simulink model "section4_simulation_editedbyzym"  (R2023b)
settings: Solver=FixedStepAuto  StartTime=0.0  StopTime=620  FixedStep=0.001  RelTol=1e-3
(part 1 of 2)
settings Model: PacingRate=100  Creator=DELL  LastModifiedBy=Administrator
settings SolverCC: AlgebraicLoopSolver=TrustRegion
settings OptimizationCC: EnhancedBackFolding=on  PassReuseOutputArgsThreshold=0  MaxStackSize=64  OptimizeBlockOrder=speed  DifferentSizesBufferReuse=on  OptimizationCustomize=off
settings DebuggingCC: ParameterTunabilityLossMsg=error  UnconnectedInputMsg=warning  UnconnectedOutputMsg=warning  UnconnectedLineMsg=warning  ArithmeticOperatorsInVariantConditions=warning
settings HardwareCC: ProdBitPerPointer=32  ProdBitPerSizeT=32  ProdBitPerPtrDiffT=32  ProdLargestAtomicFloat=None  ProdIntDivRoundTo=Undefined  ProdEndianess=Unspecified  ProdWordSize=32  ProdHWDeviceType=Generic->Unspecified (assume 32-bit Generic)
settings ModelReferenceCC: EnableRefExpFcnMdlSchedulingChecks=on
settings SFSimCC: MATLABDynamicMemAlloc=off  CustomCodeUndefinedFunction=UseInterfaceOnly
settings RTWCC: Toolchain=Catkin
settings CodeAppCC: ForceParamTrailComments=on  OperatorAnnotations=on
settings GRTTargetCC: TargetLangStandard=C89/C90 (ANSI)

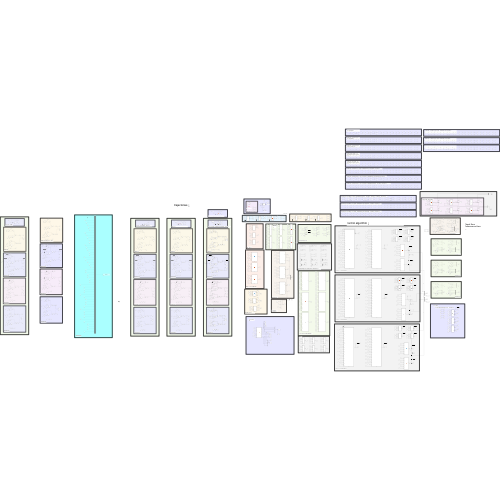
[thumbnail: Simulink's stored preview of the top-level diagram]
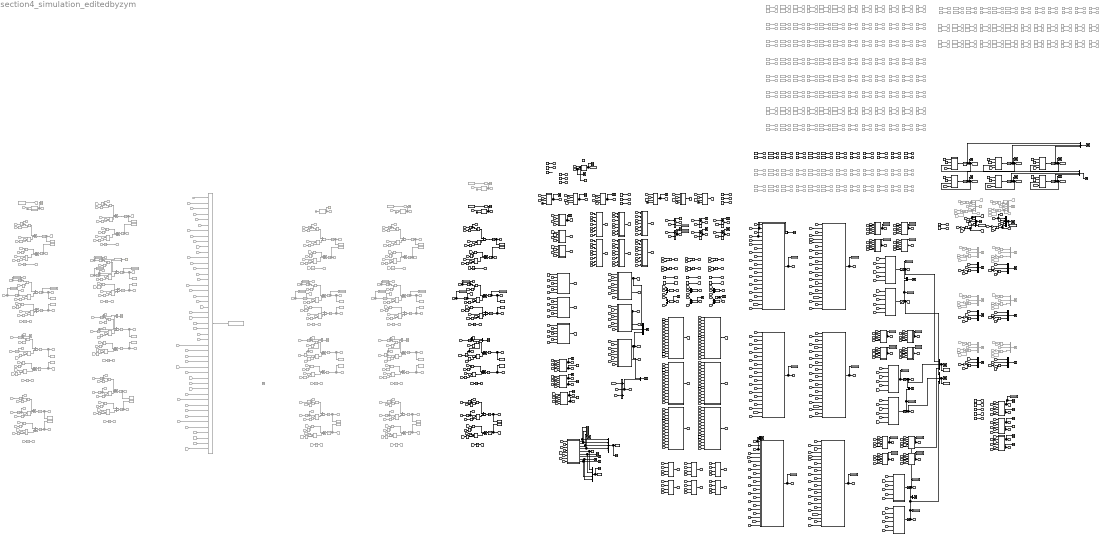
== system section4_simulation_editedbyzym ==
  note: 自适应律（6字工况）
  note: 一元二次方程中tauL和tauR的系数
  note: 控制器参数（ 固定rphi23，步长0.001,3车撞界且角度误差有稳态误差 ）
  note: dotz √
  note: 反步法新建误差delta1和delta2 √
  note: dot ei
      | √
  note: z(t)=e(t)/rou(t),并给出z(t)的上限及下限的绝对值 √
  note: 动力学模块
  note: rPHIji
  note: rdji
  note: ei 距离和角度误差√
  note: phiji,arfji（4.5）√
  note: dji（4.5）√
  note: dot,dji 三个从车的dji导数√
  note: dot,arfji,phiji √
  note: 控制器设计（1）Controller of Robot 1
  note: 预设性能对比1
  note: 预设性能对比2
  note: 预设性能对比3
  note: 预设性能对比
  note: Toworkspace
  note: 小车的转动惯量用圆柱模型来估算；J=1/2*M*L^2
  note: 我猜是队形设置，即理想间距和角度
      | 原文中（3.71）
  note: rphi23由计算得到（4.5）
  note: 为何dphi23有一个额外的修正？
  note: 编队距离和角度参数
  note: 预设性能函数
  note: 控制器设计（2） Controller of Robot 2
  note: 控制器设计（3） Controller of Robot 3
  note: leader运动学模型 原文（2.6）
  note: follower1模型
  note: follower3模型
  note: follower2模型
  note: 控制器参数（步长0.001,3车撞界且角度误差有稳态误差）
  note: follower3模型
  note: follower1模型
  note: follower2模型
  note: leader模型
  note: 6字型工况（调试）
  note: 控制器参数(固定rphi23，步长0.001,3车撞界且角度误差有稳态误差)
  note: follower3模型
  note: follower1模型
  note: follower2模型
  note: leader模型
  note: 6字工况改丝带工况t=620（从直线调试，成功运行）
  note: 控制器参数（步长0.001,直线工况收敛，lowz3p=20）
  note: 控制器参数（步长0.001,直线工况收敛，lowz3p=50）
  note: 控制器参数（步长0.001,直线工况收敛，lowz3p=50,力矩双向限幅10）
  note: 控制器参数（步长0.001,直线工况收敛，lowz3p=50,力矩双向限幅5）
  note: 控制器参数（步长0.001,直线工况收敛，lowz3p=50,力矩双向限幅2.5）
  note: 控制器参数（步长0.001,直线工况、6字工况收敛较好，lowz3p=50,3车力矩双向限幅2.5，带初始误差）
  note: follower3模型
  note: follower1模型
  note: follower2模型
  note: leader模型
  note: a 型工况 （从直线调试，成功运行）
  note: 控制器参数（步长0.001,α工况工况收敛，lowz3p=50,3车力矩双向限幅2.5，带初始误差）
  note: 控制器参数（步长0.001,α工况工况收敛，lowz3p=50,3车力矩双向限幅1.5，1,2车限幅1，带初始误差）
  note: 控制器参数（步长0.001,6字工况收敛，lowz3p=50,3车限幅1.5，1,2车限幅1，带初始误差，控制器修正，带自适应律）
  note: 控制器参数（步长0.001,直线工况、6字工况收敛较好，lowz3p=50,3车限幅1.5，1,2车限幅1，带初始误差）
  note: 控制器参数（步长0.001,α工况工况收敛，lowz3p=50,3车力矩双向限幅2.5，1,2车限幅1，带初始误差）
  note: 6字工况（从直线调试，成功运行）
  note: follower3模型
  note: follower1模型
  note: follower2模型
  note: leader模型
  note: 实验工况
  note: Check Error Performance Here
      | ←
  note: control algorithm ↓
  note: trajectories ↓
  " " : Integrator  Commented=on  InitialCondition=pi/7
  -1 : Integrator  Commented=on  InitialCondition=-25
  -14→-1 : Integrator  Commented=on  InitialCondition=-14
  -14→-3 : Integrator  Commented=on  InitialCondition=-25
  -25 : Integrator  InitialCondition=-25
  -3→1 : Integrator  Commented=on  InitialCondition=-1
  -3→2 : Integrator
  -3→3 : Integrator  Commented=on
  -3→4 : Integrator  Commented=on
  -8.1 : Integrator  Commented=on  InitialCondition=-10
  -8.66025 : Integrator  InitialCondition=-10
  Add : Sum  Inputs=+-+
  Add{1..4,12,14,33,35,43,45} (10 alike) : Sum  Inputs=+-
  Add{6,8,10,13,17,19,21,23,26,28,30,32,48,50,52,54} (16 alike) : Sum  Commented=on
  Add{5,7,9,11,18,20,22,24..25,27,29,31,47,49,51,53} (16 alike) : Sum  Commented=on  Inputs=+-
  Add{34,42,44,46} (4 alike) : Sum
  Clock{,1..3,6..7,9} (7 alike) : Clock
      Clock settings: Decimation=100
      Clock2 settings: Decimation=100
  Clock{4..5,8,10,19} (5 alike) : Clock  Commented=on
  Constant : Constant  Value=0.2
  Constant{1..2,5,7,17,24,35,38..43,69..72,76..77,90..94,98,100,113..116,119..120,122,136..137,139..140,148..149,162..166,169,182..185,188..189,202..205,208..209,222..225,228..229,242..245,248,251,284,297..300,303,306,313,316,318..321,325} (83 alike) : Constant  Commented=on
  Constant{10..11,63,129,156,167,176,186,196,206,216,226,234,236,249..250,289,291,301,308,324} (21 alike) : Constant  Commented=on  Value=0.001
  Constant{18..19,23,36..37,45,57..58,67..68,78..79,83,88..89,95,101..102,106,111..112,117,123..124,134..135,150..151,160..161,170..171,180..181,190..191,200..201,210..211,230..231,285..286} (44 alike) : Constant  Commented=on  Value=10
  Constant{6,20,59,80,103,125,152,172,192,212,232,287,322} (13 alike) : Constant  Commented=on  Value=0.2
  Constant{8,21,60,81,104,126,153,173,193,213,233,288,323} (13 alike) : Constant  Commented=on  Value=0.09
  Constant105 : Constant  Commented=on  Value=2.5
  Constant{13,25,29,62,65,75,84,86,107,109,128,131,154,158,178,198,218,238,293,310} (20 alike) : Constant  Commented=on  Value=0.0001
  Constant{12,26,64,85,108,127,130,157,177,197,217,237,292,309} (14 alike) : Constant  Commented=on  Value=0.005
  Constant{30,66,87,110,132,159,168,179,187,199,207,227,247,302,315} (15 alike) : Constant  Commented=on  Value=0.1
  Constant118 : Constant  Commented=on  Value=2
  Constant121 : Constant  Value=50
  Constant133 : Constant  Value=-pi/6
  Constant138 : Constant  Value=pi/6
  Constant{14,56,97,143,174,219,239,246,294,311,314} (11 alike) : Constant  Commented=on  Value=0.01
  Constant141 : Constant  Commented=on  Value=50
  Constant142 : Constant  Commented=on  Value=0.0064
  Constant{144,263..264,275} (4 alike) : Constant  Value=5
  Constant{28,145,257,277,281,283} (6 alike) : Constant  Value=0.1
  Constant146 : Constant  Value=0.25
  Constant147 : Constant  Value=0.16
  Constant{15,34,220..221,240..241,290,295..296,312,317} (11 alike) : Constant  Commented=on  Value=5
  Constant155 : Constant  Commented=on  Value=50
  Constant175 : Constant  Commented=on  Value=9
  Constant194 : Constant  Commented=on  Value=0.009
  Constant195 : Constant  Commented=on  Value=20
  Constant214 : Constant  Commented=on  Value=0.009
  Constant215 : Constant  Commented=on  Value=20
  Constant22 : Constant  Commented=on  Value=2.5
  Constant235 : Constant  Commented=on  Value=0.5
  Constant{46,50..54,252,265..268,271..273,276,278..279,282,304..305} (20 alike) : Constant
  Constant{3..4,31,253..254} (5 alike) : Constant  Value=10
  Constant255 : Constant  Value=0.2
  Constant256 : Constant  Value=0.09
  Constant{258,269..270,280} (4 alike) : Constant  Value=0.001
  Constant259 : Constant  Value=0.0001
  Constant260 : Constant  Value=0.005
  Constant261 : Constant  Value=0.0001
  Constant262 : Constant  Value=0.09
  Constant27 : Constant  Value=0.06
  Constant274 : Constant  Value=0.005
  Constant307 : Constant  Commented=on  Value=0.5
  Constant32 : Constant  Value=-pi/6
  Constant33 : Constant  Value=12
  Constant44 : Constant  Value=-0.38
  Constant47 : Constant  Value=0.06
  Constant48 : Constant  Value=0.03
  Constant49 : Constant  Value=0.6
  Constant55 : Constant  Commented=on  Value=2
  Constant61 : Constant  Commented=on  Value=0.0101
  Constant73 : Constant  Commented=on  Value=50
  Constant74 : Constant  Commented=on  Value=0.00005
  Constant82 : Constant  Commented=on  Value=2.5
  Constant9 : Constant  Commented=on  Value=0.5
  Constant96 : Constant  Commented=on  Value=0.8
  Constant99 : Constant  Commented=on  Value=0.0000698
  Cos{1,3,5,7,12,14,16,18..19,21,23,25,41,43,45,47} (16 alike) : Trigonometry  Commented=on  Operator=cos
  Cos{2,4,6,8,11,13,15,17,20,22,24,26,42,44,46,48} (16 alike) : Trigonometry  Commented=on
  Cos{27,35,37,39} (4 alike) : Trigonometry  Operator=cos
  Cos{34,36,38,40} (4 alike) : Trigonometry
  Didm_hat : Scope
  Dipm_hat : Scope
  Display{1..8,12..29,36..38,41} (30 alike) : Display
  Display{9..11,30..35,39..40,42} (12 alike) : Display  Commented=on
  Divide{,1..5} (6 alike) : Product  Inputs=*/  RndMeth=Zero  SaturateOnIntegerOverflow=on
  Fcn : Fcn  Expr=(u(2)-u(3))/(u(3)-u(1))
  Fcn1 : Fcn  Expr=(u(2)-u(3))/(u(3)-u(1))
  Fcn2 : Fcn  Expr=(u(2)-u(3))/(u(3)-u(1))
  Fcn3 : Fcn  Expr=(u(1)+u(2))/(u(1)-u(2))
  Fcn4 : Fcn  Expr=(u(1)+u(2))/(u(1)-u(2))
  Fcn5 : Fcn  Expr=(u(1)+u(2))/(u(1)-u(2))
  From{134,344,858,950} (4 alike) : From  Commented=on  GotoTag=dvL
  From{136,345,859,951} (4 alike) : From  Commented=on  GotoTag=dv1
  From{137,346,860,952} (4 alike) : From  Commented=on  GotoTag=domg1
  From{139,143,159,163,241,246,270,276,347,351,825,829,835,839,844,853,861,865,871,875,881,885,890,896,953,961,967,971,977,981,986,992} (32 alike) : From  Commented=on  GotoTag=h  TagVisibility=global
  From{140,144..146,348,352..354,716,862,866..868,954,962..964} (17 alike) : From  Commented=on  GotoTag=theta1  TagVisibility=global
  From{141,349,712,863,955} (5 alike) : From  Commented=on  GotoTag=v1  TagVisibility=global
  From{142,269,350,713,843,864,889,956,985} (9 alike) : From  Commented=on  GotoTag=omg1  TagVisibility=global
  From{147,355,869,965} (4 alike) : From  Commented=on  GotoTag=dv2
  From{156,824,870,966} (4 alike) : From  Commented=on  GotoTag=domg2
  From{160,164..166,709,826,830..832,872,876..878,968,972..974} (17 alike) : From  Commented=on  GotoTag=theta2  TagVisibility=global
  From{161,710,827,873,969} (5 alike) : From  Commented=on  GotoTag=v2  TagVisibility=global
  From{162,271,711,828,845,874,891,970,987} (9 alike) : From  Commented=on  GotoTag=omg2  TagVisibility=global
  From{167,833,879,975} (4 alike) : From  Commented=on  GotoTag=dv3
  From2 : From  Commented=on  GotoTag=ks
  From{208,834,880,976} (4 alike) : From  Commented=on  GotoTag=domg3
  From218 : From  Commented=on  GotoTag=S2d
  From{219..220,365..366,397..398,505..506} (8 alike) : From  Commented=on  GotoTag=roud  TagVisibility=global
  From221 : From  Commented=on  GotoTag=ksd2
  From222 : From  Commented=on  GotoTag=S2p
  From{223..224,369..370,401..402,611..612} (8 alike) : From  Commented=on  GotoTag=roup  TagVisibility=global
  From225 : From  Commented=on  GotoTag=ksd2
  From226 : From  Commented=on  GotoTag=ked2
  From227 : From  Commented=on  GotoTag=ksp2
  From228 : From  Commented=on  GotoTag=ksp2
  From235 : From  Commented=on  GotoTag=kep2
  From{242,247,251..252,721,836,840..842,882,886..888,978,982..984} (17 alike) : From  Commented=on  GotoTag=theta3  TagVisibility=global
  From{243,724,837,883,979} (5 alike) : From  Commented=on  GotoTag=v3  TagVisibility=global
  From{245,272,725,838,846,884,892,980,988} (9 alike) : From  Commented=on  GotoTag=omg3  TagVisibility=global
  From{273,277,279,281,704,847,854..856,893,897,899,901,989,994,996,998} (17 alike) : From  Commented=on  GotoTag=thetaL  TagVisibility=global
  From{274,705,851,894,990} (5 alike) : From  Commented=on  GotoTag=vL  TagVisibility=global
  From{275,278,282,706,852,857,895,898,902,991,995,999} (12 alike) : From  Commented=on  GotoTag=omgL  TagVisibility=global
  From280 : From  Commented=on  GotoTag=ks
  From364 : From  Commented=on  GotoTag=S3d
  From367 : From  Commented=on  GotoTag=ksd3
  From368 : From  Commented=on  GotoTag=S3p
  From371 : From  Commented=on  GotoTag=ksd3
  From372 : From  Commented=on  GotoTag=ked3
  From373 : From  Commented=on  GotoTag=ksp3
  From374 : From  Commented=on  GotoTag=ksp3
  From375 : From  Commented=on  GotoTag=kep3
  From396 : From  Commented=on  GotoTag=S1d  TagVisibility=global
  From{399,403,507,613} (4 alike) : From  Commented=on  GotoTag=ksd1  TagVisibility=global
  From400 : From  Commented=on  GotoTag=S1p  TagVisibility=global
  From404 : From  Commented=on  GotoTag=ked
  From{405..406,615..616} (4 alike) : From  Commented=on  GotoTag=ksp1
  From407 : From  Commented=on  GotoTag=kep
  From408 : From  Commented=on  GotoTag=S2d  TagVisibility=global
  From415 : From  Commented=on  GotoTag=S3d  TagVisibility=global
  From416 : From  Commented=on  GotoTag=S2p  TagVisibility=global
  From417 : From  Commented=on  GotoTag=S3p  TagVisibility=global
  From462角速度1 : From  Commented=on  GotoTag=omgL  TagVisibility=global
  From504 : From  Commented=on  GotoTag=S1d  TagVisibility=global
  From610 : From  Commented=on  GotoTag=S1p  TagVisibility=global
  From614 : From  Commented=on  GotoTag=ked
  From617 : From  Commented=on  GotoTag=kep
  From683 : From  Commented=on  GotoTag=xL  TagVisibility=global
  From703 : From  Commented=on  GotoTag=yL  TagVisibility=global
  From707 : From  Commented=on  GotoTag=x2  TagVisibility=global
  From708 : From  Commented=on  GotoTag=y2  TagVisibility=global
  From714 : From  Commented=on  GotoTag=x1  TagVisibility=global
  From715 : From  Commented=on  GotoTag=y1  TagVisibility=global
  From717 : From  Commented=on  GotoTag=tr1  TagVisibility=global
  From718 : From  Commented=on  GotoTag=tl1  TagVisibility=global
  From719 : From  Commented=on  GotoTag=tr2  TagVisibility=global
  From720 : From  Commented=on  GotoTag=tl2  TagVisibility=global
  From722 : From  Commented=on  GotoTag=y3  TagVisibility=global
  From723 : From  Commented=on  GotoTag=x3  TagVisibility=global
  From726 : From  Commented=on  GotoTag=tr3  TagVisibility=global
  From727 : From  Commented=on  GotoTag=tl3  TagVisibility=global
  From728 : From  Commented=on  GotoTag=S1d  TagVisibility=global
  From729 : From  Commented=on  GotoTag=S1p  TagVisibility=global
  From730 : From  Commented=on  GotoTag=e1d
  From731 : From  Commented=on  GotoTag=e1p
  From732 : From  Commented=on  GotoTag=S2d  TagVisibility=global
  From733 : From  Commented=on  GotoTag=S2p  TagVisibility=global
  From734 : From  Commented=on  GotoTag=e2d
  From735 : From  Commented=on  GotoTag=e2p
  From736 : From  Commented=on  GotoTag=S3d  TagVisibility=global
  From737 : From  Commented=on  GotoTag=S3p  TagVisibility=global
  From739 : From  Commented=on  GotoTag=e3p
  From740 : From  Commented=on  GotoTag=Supd
  From741 : From  Commented=on  GotoTag=Sdod
  From742 : From  Commented=on  GotoTag=Supp
  From743 : From  Commented=on  GotoTag=Sdop
  From744 : From  Commented=on  GotoTag=eupd
  From745 : From  Commented=on  GotoTag=edod
  From746 : From  Commented=on  GotoTag=eupp
  From747 : From  Commented=on  GotoTag=edop
  From774 : From  Commented=on  GotoTag=e3d
  From900 : From  Commented=on  GotoTag=ks
  Gain{,1,4..5,8..9,12..13} (8 alike) : Gain  Gain=-1
  Gain{2..3,6..7,10..11,14..15} (8 alike) : Gain  Commented=on  Gain=-1
  Goto{1,127,133,218,240,303,305,350,374,398,422,446,488} (13 alike) : Goto  Commented=on  GotoTag=k2d
  Goto{10,174,198,246,311,332,356,380,404,428,452,496,514} (13 alike) : Goto  Commented=on  GotoTag=k2ed
  Goto106 : Goto  Commented=on  GotoTag=Supd
  Goto107 : Goto  Commented=on  GotoTag=Sdod
  Goto108 : Goto  Commented=on  GotoTag=Supp
  Goto109 : Goto  Commented=on  GotoTag=Sdop
  Goto{11,175,247,289,312,333,357,381,405,429,453,497,515} (13 alike) : Goto  Commented=on  GotoTag=k1ed
  Goto{12,176,248,290,313,334,358,382,406,430,454,498,516} (13 alike) : Goto  Commented=on  GotoTag=k3ed
  Goto{38,52,122,259,324,345,369,393,417,441,465,509,527} (13 alike) : Goto  Commented=on  GotoTag=k1roud
  Goto{39,53,123,260,325,346,370,394,418,442,466,510,528} (13 alike) : Goto  Commented=on  GotoTag=k3roud
  Goto{40,54,124,261,326,347,371,395,419,443,467,511,529} (13 alike) : Goto  Commented=on  GotoTag=k2roup
  Goto{41,55,125,262,327,348,372,396,420,444,468,512,530} (13 alike) : Goto  Commented=on  GotoTag=k1roup
  Goto{42,56,126,263,328,349,373,397,421,445,469,513,531} (13 alike) : Goto  Commented=on  GotoTag=k3roup
  Goto{5,128,134,219,241,306,351,375,399,423,447,491,532} (13 alike) : Goto  Commented=on  GotoTag=k2p
  Goto{6,129,170,220,242,307,352,376,400,424,448,492,533} (13 alike) : Goto  Commented=on  GotoTag=k1d
  Goto{13,177,249,291,314,335,359,383,407,431,455,499,517} (13 alike) : Goto  Commented=on  GotoTag=D2dm
  Goto{7,130,171,243,308,329,353,377,401,425,449,493,534} (13 alike) : Goto  Commented=on  GotoTag=k1p
  Goto{8,131,172,244,309,330,354,378,402,426,450,494,535} (13 alike) : Goto  Commented=on  GotoTag=k3d
  Goto{9,132,173,245,310,331,355,379,403,427,451,495,536} (13 alike) : Goto  Commented=on  GotoTag=k3p
  Goto{14,178,250,292,315,336,360,384,408,432,456,500,518} (13 alike) : Goto  Commented=on  GotoTag=D2pm
  Goto{15,179,251,293,316,337,361,385,409,433,457,501,519} (13 alike) : Goto  Commented=on  GotoTag=D1dm
  Goto{24,180,252,294,317,338,362,386,410,434,458,502,520} (13 alike) : Goto  Commented=on  GotoTag=D1pm
  Goto{29,181,253,295,318,339,363,387,411,435,459,503,521} (13 alike) : Goto  Commented=on  GotoTag=D3dm
  Goto{33,182,254,296,319,340,364,388,412,436,460,504,522} (13 alike) : Goto  Commented=on  GotoTag=D3pm
  Goto{34,189,255,297,320,341,365,389,413,437,461,505,523} (13 alike) : Goto  Commented=on  GotoTag=k2ep
  Goto{35,190,256,298,321,342,366,390,414,438,462,506,524} (13 alike) : Goto  Commented=on  GotoTag=k1ep
  Goto{36,191,257,299,322,343,367,391,415,439,463,507,525} (13 alike) : Goto  Commented=on  GotoTag=k3ep
  Goto{221,264,489,566} (4 alike) : Goto  Commented=on  GotoTag=xL  TagVisibility=global
  Goto{222,265,490,567} (4 alike) : Goto  Commented=on  GotoTag=vL  TagVisibility=global
  Goto{223,266,470,547} (4 alike) : Goto  Commented=on  GotoTag=yL  TagVisibility=global
  Goto{224,267,471,548} (4 alike) : Goto  Commented=on  GotoTag=thetaL  TagVisibility=global
  Goto{225,272,473,550} (4 alike) : Goto  Commented=on  GotoTag=x1  TagVisibility=global
  Goto{226,273,474,551} (4 alike) : Goto  Commented=on  GotoTag=v1  TagVisibility=global
  Goto{227,274,475,552} (4 alike) : Goto  Commented=on  GotoTag=omg1  TagVisibility=global
  Goto{228,275,476,553} (4 alike) : Goto  Commented=on  GotoTag=y1  TagVisibility=global
  Goto{229,276,477,554} (4 alike) : Goto  Commented=on  GotoTag=x2  TagVisibility=global
  Goto{230,277,478,555} (4 alike) : Goto  Commented=on  GotoTag=v2  TagVisibility=global
  Goto{231,278,479,556} (4 alike) : Goto  Commented=on  GotoTag=omg2  TagVisibility=global
  Goto{232,281,480,557} (4 alike) : Goto  Commented=on  GotoTag=y2  TagVisibility=global
  Goto{233,282,481,558} (4 alike) : Goto  Commented=on  GotoTag=x3  TagVisibility=global
  Goto{234,283,482,559} (4 alike) : Goto  Commented=on  GotoTag=v3  TagVisibility=global
  Goto{235,284,483,560} (4 alike) : Goto  Commented=on  GotoTag=omg3  TagVisibility=global
  Goto{236,285,484,561} (4 alike) : Goto  Commented=on  GotoTag=y3  TagVisibility=global
  Goto{237,286,485,562} (4 alike) : Goto  Commented=on  GotoTag=theta1  TagVisibility=global
  Goto{238,287,486,563} (4 alike) : Goto  Commented=on  GotoTag=theta2  TagVisibility=global
  Goto{239,288,487,564} (4 alike) : Goto  Commented=on  GotoTag=theta3  TagVisibility=global
  Goto{37,51,258,300,323,344,368,392,416,440,464,508,526} (13 alike) : Goto  Commented=on  GotoTag=k2roud
  Goto{270,472,537,549} (4 alike) : Goto  Commented=on  GotoTag=omgL  TagVisibility=global
  Goto304 : Goto  Commented=on  GotoTag=ks
  Goto538 : Goto  Commented=on  GotoTag=ks
  Goto565 : Goto  Commented=on  GotoTag=ks
  Integrator : Integrator  InitialCondition=10
  Integrator1 : Integrator  InitialCondition=5
  Integrator{9..10,14..15,18,30..31,35,38..40,49,56..57,64..65,68,90..91,96..97,100} (22 alike) : Integrator  Commented=on
  Integrator{17,19,33,67,69,99,101} (7 alike) : Integrator  Commented=on  InitialCondition=0.6
  Integrator102 : Integrator  Commented=on  InitialCondition=pi/6
  Integrator11 : Integrator  Commented=on  InitialCondition=5
  Integrator12 : Integrator  Commented=on  InitialCondition=13
  Integrator{7,13,28,41..42,53,62,88,94} (9 alike) : Integrator  Commented=on  InitialCondition=0.5
  Integrator16 : Integrator  Commented=on  InitialCondition=-2
  Integrator2 : Integrator  InitialCondition=0.5
  Integrator20 : Integrator  Commented=on  InitialCondition=pi/6
  Integrator26 : Integrator  Commented=on  InitialCondition=85
  Integrator27 : Integrator  Commented=on  InitialCondition=91
  Integrator29 : Integrator  Commented=on  InitialCondition=12
  Integrator3 : Integrator  InitialCondition=10
  Integrator32 : Integrator  Commented=on  InitialCondition=79
  Integrator34 : Integrator  Commented=on  InitialCondition=4
  Integrator36 : Integrator  Commented=on  InitialCondition=85
  Integrator4 : Integrator  InitialCondition=5
  Integrator43 : Integrator  Commented=on  InitialCondition=12
  Integrator45 : Integrator  Commented=on  InitialCondition=20
  Integrator5 : Integrator  InitialCondition=10
  Integrator51 : Integrator  Commented=on  InitialCondition=1
  Integrator55 : Integrator  Commented=on  InitialCondition=-8
  Integrator6 : Integrator  Commented=on  InitialCondition=1
  Integrator60 : Integrator  Commented=on  InitialCondition=5
  Integrator61 : Integrator  Commented=on  InitialCondition=13
  Integrator63 : Integrator  Commented=on  InitialCondition=-9
  Integrator66 : Integrator  Commented=on  InitialCondition=-3
  Integrator70 : Integrator  Commented=on  InitialCondition=pi/9
  Integrator71 : Integrator  InitialCondition=1
  Integrator72 : Integrator  InitialCondition=0.5
  Integrator73 : Integrator  InitialCondition=-8
  Integrator{74..75,80..81,84} (5 alike) : Integrator
  Integrator76 : Integrator  InitialCondition=5
  Integrator77 : Integrator  InitialCondition=13
  Integrator78 : Integrator  InitialCondition=0.5
  Integrator8 : Integrator  Commented=on  InitialCondition=-8
  Integrator82 : Integrator  InitialCondition=-2
  Integrator83 : Integrator  InitialCondition=0.6
  Integrator85 : Integrator  InitialCondition=0.6
  Integrator86 : Integrator  InitialCondition=pi/6
  Integrator87 : Integrator  Commented=on  InitialCondition=1
  Integrator89 : Integrator  Commented=on  InitialCondition=-8
  Integrator92 : Integrator  Commented=on  InitialCondition=5
  Integrator93 : Integrator  Commented=on  InitialCondition=13
  Integrator95 : Integrator  Commented=on  InitialCondition=-8.66025
  Integrator98 : Integrator  Commented=on  InitialCondition=-2
  MATLAB Function : MATLAB Function  TreatAsAtomicUnit=on
  MATLAB Function1 : MATLAB Function  TreatAsAtomicUnit=on
  MATLAB Function10 : MATLAB Function  TreatAsAtomicUnit=on
  MATLAB Function11 : MATLAB Function  TreatAsAtomicUnit=on
  MATLAB Function12 : MATLAB Function  TreatAsAtomicUnit=on
  MATLAB Function13 : MATLAB Function  TreatAsAtomicUnit=on
  MATLAB Function14 : MATLAB Function  TreatAsAtomicUnit=on
  MATLAB Function15 : MATLAB Function  TreatAsAtomicUnit=on
  MATLAB Function16 : MATLAB Function  Commented=on  TreatAsAtomicUnit=on
  MATLAB Function17 : MATLAB Function  TreatAsAtomicUnit=on
  MATLAB Function18 : MATLAB Function  TreatAsAtomicUnit=on
  MATLAB Function19 : MATLAB Function  TreatAsAtomicUnit=on
  MATLAB Function2 : MATLAB Function  TreatAsAtomicUnit=on
  MATLAB Function20 : MATLAB Function  TreatAsAtomicUnit=on
  MATLAB Function21 : MATLAB Function  TreatAsAtomicUnit=on
  MATLAB Function22 : MATLAB Function  TreatAsAtomicUnit=on
  MATLAB Function23 : MATLAB Function  TreatAsAtomicUnit=on
  MATLAB Function24 : MATLAB Function  TreatAsAtomicUnit=on
  MATLAB Function25 : MATLAB Function  TreatAsAtomicUnit=on
  MATLAB Function26 : MATLAB Function  TreatAsAtomicUnit=on
  MATLAB Function27 : MATLAB Function  TreatAsAtomicUnit=on
  MATLAB Function28 : MATLAB Function  TreatAsAtomicUnit=on
  MATLAB Function29 : MATLAB Function  TreatAsAtomicUnit=on
  MATLAB Function3 : MATLAB Function  TreatAsAtomicUnit=on
  MATLAB Function30 : MATLAB Function  TreatAsAtomicUnit=on
  MATLAB Function31 : MATLAB Function  TreatAsAtomicUnit=on
  MATLAB Function32 : MATLAB Function  TreatAsAtomicUnit=on
  MATLAB Function33 : MATLAB Function  TreatAsAtomicUnit=on
  MATLAB Function34 : MATLAB Function  TreatAsAtomicUnit=on
  MATLAB Function35 : MATLAB Function  TreatAsAtomicUnit=on
  MATLAB Function36 : MATLAB Function  TreatAsAtomicUnit=on
  MATLAB Function37 : MATLAB Function  Commented=on  TreatAsAtomicUnit=on
  MATLAB Function38 : MATLAB Function  Commented=on  TreatAsAtomicUnit=on
  MATLAB Function4 : MATLAB Function  TreatAsAtomicUnit=on
  MATLAB Function5 : MATLAB Function  TreatAsAtomicUnit=on
  MATLAB Function6 : MATLAB Function  TreatAsAtomicUnit=on
  MATLAB Function7 : MATLAB Function  TreatAsAtomicUnit=on
  MATLAB Function8 : MATLAB Function  TreatAsAtomicUnit=on
  MATLAB Function9 : MATLAB Function  TreatAsAtomicUnit=on
  Manual Switch : ManualSwitch  Commented=on  CurrentSetting=0
  Mux{,1..2,5..6,13..14,26,28,31..33,48..49} (14 alike) : Mux  Inputs=3
  Mux10 : Mux  Inputs=5
  Mux11 : Mux  Commented=on  Inputs=5
  Mux12 : Mux  Commented=on  Inputs=5
  Mux{15..16,18..23,27,29} (10 alike) : Mux  Inputs=2
  Mux17 : Mux  Commented=on  Inputs=47
  Mux{24..25,30,34} (4 alike) : Mux  Commented=on  Inputs=2
  Mux{3..4,7..8,50..51} (6 alike) : Mux  Commented=on  Inputs=3
  Mux63 : Mux
  Mux78 : Mux
  Mux9 : Mux  Inputs=5
  Product{1..3,5..6,12..13,17..18,24..25,28..29,32,39..41,44..45,48..49,52,55..57,60..61,64..65,68,87..89,92..93,98..99,102,105..106} (40 alike) : Product  Commented=on  Inputs=3
  Product{9..11,16,21..22,74..75,78..79,82..83,85..86,95..96} (16 alike) : Product
  Product{4,7..8,14..15,19..20,23,26..27,30..31,33..34,42..43,46..47,50..51,53..54,58..59,62..63,66..67,69..70,90..91,94,97,100..101,103..104,107..108} (40 alike) : Product  Commented=on
  Product{71..73,76..77,80..81,84} (8 alike) : Product  Inputs=3
  Saturation{6..11} (6 alike) : Saturate  UpperLimit=1  LowerLimit=-1
  Scope{,1..11,14..17,24..34,39..50,53..56,58,60..61,66..70,81..82,99..108} (63 alike) : Scope
  Scope{12..13,18..22,35..36,51..52,57,59,62..63,71..72} (17 alike) : Scope  Commented=on
  Sin{1,3,5,7,18,20,22,24..25,27,29,31,41,43,45,47} (16 alike) : Trigonometry  Commented=on
  Sin{2,4,6,8,17,19,21,23,26,28,30,32,42,44,46,48} (16 alike) : Trigonometry  Commented=on  Operator=cos
  Sin{33,35,37,39} (4 alike) : Trigonometry
  Sin{34,36,38,40} (4 alike) : Trigonometry  Operator=cos
  To Workspace : ToWorkspace  VariableName=ed  SampleTime=-1
      settings: Save2DSignal=2-D array (concatenate along first dimension)
  To Workspace1 : ToWorkspace  Commented=on  VariableName=x1  SampleTime=-1
      settings: Save2DSignal=2-D array (concatenate along first dimension)
  To Workspace10 : ToWorkspace  VariableName=tauiL  SampleTime=-1
      settings: Save2DSignal=2-D array (concatenate along first dimension)
  To Workspace11 : ToWorkspace  VariableName=tauiR  SampleTime=-1
      settings: Save2DSignal=2-D array (concatenate along first dimension)
  To Workspace13 : ToWorkspace  VariableName=bianchang  SampleTime=-1
      settings: Save2DSignal=2-D array (concatenate along first dimension)
  To Workspace15 : ToWorkspace  VariableName=JIAO  SampleTime=-1
      settings: Save2DSignal=2-D array (concatenate along first dimension)
  To Workspace18 : ToWorkspace  Commented=on  VariableName=xL1  SampleTime=-1
      settings: Save2DSignal=2-D array (concatenate along first dimension)
  To Workspace19 : ToWorkspace  Commented=on  VariableName=yL1  SampleTime=-1
      settings: Save2DSignal=2-D array (concatenate along first dimension)
  To Workspace2 : ToWorkspace  Commented=on  VariableName=y1  SampleTime=-1
      settings: Save2DSignal=2-D array (concatenate along first dimension)
  To Workspace20 : ToWorkspace  Commented=on  VariableName=x  SampleTime=-1
      settings: Save2DSignal=2-D array (concatenate along first dimension)
  To Workspace21 : ToWorkspace  Commented=on  VariableName=y  SampleTime=-1
      settings: Save2DSignal=2-D array (concatenate along first dimension)
  To Workspace22 : ToWorkspace  Commented=on  VariableName=x4  SampleTime=-1
      settings: Save2DSignal=2-D array (concatenate along first dimension)
  To Workspace23 : ToWorkspace  Commented=on  VariableName=y4  SampleTime=-1
      settings: Save2DSignal=2-D array (concatenate along first dimension)
  To Workspace24 : ToWorkspace  Commented=on  VariableName=x5  SampleTime=-1
      settings: Save2DSignal=2-D array (concatenate along first dimension)
  To Workspace25 : ToWorkspace  Commented=on  VariableName=y5  SampleTime=-1
      settings: Save2DSignal=2-D array (concatenate along first dimension)
  To Workspace26 : ToWorkspace  Commented=on  VariableName=x6  SampleTime=-1
      settings: Save2DSignal=2-D array (concatenate along first dimension)
  To Workspace27 : ToWorkspace  Commented=on  VariableName=y6  SampleTime=-1
      settings: Save2DSignal=2-D array (concatenate along first dimension)
  To Workspace28 : ToWorkspace  Commented=on  VariableName=xL2  SampleTime=-1
      settings: Save2DSignal=2-D array (concatenate along first dimension)
  To Workspace29 : ToWorkspace  Commented=on  VariableName=yL2  SampleTime=-1
      settings: Save2DSignal=2-D array (concatenate along first dimension)
  To Workspace3 : ToWorkspace  Commented=on  VariableName=xL  SampleTime=-1
      settings: Save2DSignal=2-D array (concatenate along first dimension)
  To Workspace30 : ToWorkspace  Commented=on  VariableName=x7  SampleTime=-1
      settings: Save2DSignal=2-D array (concatenate along first dimension)
  To Workspace31 : ToWorkspace  Commented=on  VariableName=y7  SampleTime=-1
      settings: Save2DSignal=2-D array (concatenate along first dimension)
  To Workspace32 : ToWorkspace  Commented=on  VariableName=x8  SampleTime=-1
      settings: Save2DSignal=2-D array (concatenate along first dimension)
  To Workspace33 : ToWorkspace  Commented=on  VariableName=y8  SampleTime=-1
      settings: Save2DSignal=2-D array (concatenate along first dimension)
  To Workspace34 : ToWorkspace  VariableName=x9  SampleTime=-1
      settings: Save2DSignal=2-D array (concatenate along first dimension)
  To Workspace35 : ToWorkspace  VariableName=y9  SampleTime=-1
      settings: Save2DSignal=2-D array (concatenate along first dimension)
  To Workspace36 : ToWorkspace  VariableName=xL3  SampleTime=-1
      settings: Save2DSignal=2-D array (concatenate along first dimension)
  To Workspace37 : ToWorkspace  VariableName=yL3  SampleTime=-1
      settings: Save2DSignal=2-D array (concatenate along first dimension)
  To Workspace38 : ToWorkspace  VariableName=x10  SampleTime=-1
      settings: Save2DSignal=2-D array (concatenate along first dimension)
  To Workspace39 : ToWorkspace  VariableName=y10  SampleTime=-1
      settings: Save2DSignal=2-D array (concatenate along first dimension)
  To Workspace4 : ToWorkspace  Commented=on  VariableName=yL  SampleTime=-1
      settings: Save2DSignal=2-D array (concatenate along first dimension)
  To Workspace40 : ToWorkspace  VariableName=x11  SampleTime=-1
      settings: Save2DSignal=2-D array (concatenate along first dimension)
  To Workspace41 : ToWorkspace  VariableName=y11  SampleTime=-1
      settings: Save2DSignal=2-D array (concatenate along first dimension)
  To Workspace42 : ToWorkspace  Commented=on  VariableName=x12  SampleTime=-1
      settings: Save2DSignal=2-D array (concatenate along first dimension)
  To Workspace43 : ToWorkspace  Commented=on  VariableName=y12  SampleTime=-1
      settings: Save2DSignal=2-D array (concatenate along first dimension)
  To Workspace44 : ToWorkspace  Commented=on  VariableName=xL4  SampleTime=-1
      settings: Save2DSignal=2-D array (concatenate along first dimension)
  To Workspace45 : ToWorkspace  Commented=on  VariableName=yL4  SampleTime=-1
      settings: Save2DSignal=2-D array (concatenate along first dimension)
  To Workspace46 : ToWorkspace  Commented=on  VariableName=x13  SampleTime=-1
      settings: Save2DSignal=2-D array (concatenate along first dimension)
  To Workspace47 : ToWorkspace  Commented=on  VariableName=y13  SampleTime=-1
      settings: Save2DSignal=2-D array (concatenate along first dimension)
  To Workspace48 : ToWorkspace  Commented=on  VariableName=x14  SampleTime=-1
      settings: Save2DSignal=2-D array (concatenate along first dimension)
  To Workspace49 : ToWorkspace  Commented=on  VariableName=shiyanshuju  SampleTime=-1
      settings: Save2DSignal=2-D array (concatenate along first dimension)
  To Workspace5 : ToWorkspace  Commented=on  VariableName=x2  SampleTime=-1
      settings: Save2DSignal=2-D array (concatenate along first dimension)
  To Workspace50 : ToWorkspace  Commented=on  VariableName=y14  SampleTime=-1
      settings: Save2DSignal=2-D array (concatenate along first dimension)
  To Workspace6 : ToWorkspace  Commented=on  VariableName=y2  SampleTime=-1
      settings: Save2DSignal=2-D array (concatenate along first dimension)
  To Workspace7 : ToWorkspace  Commented=on  VariableName=x3  SampleTime=-1
      settings: Save2DSignal=2-D array (concatenate along first dimension)
  To Workspace8 : ToWorkspace  Commented=on  VariableName=y3  SampleTime=-1
      settings: Save2DSignal=2-D array (concatenate along first dimension)
  To Workspace9 : ToWorkspace  VariableName=ep  SampleTime=-1
      settings: Save2DSignal=2-D array (concatenate along first dimension)
  a : MATLAB Function  TreatAsAtomicUnit=on
  a1 : MATLAB Function  TreatAsAtomicUnit=on
  a10 : MATLAB Function  TreatAsAtomicUnit=on
  a11 : MATLAB Function  TreatAsAtomicUnit=on
  a2 : MATLAB Function  TreatAsAtomicUnit=on
  a3 : MATLAB Function  TreatAsAtomicUnit=on
  a4 : MATLAB Function  TreatAsAtomicUnit=on
  a5 : MATLAB Function  TreatAsAtomicUnit=on
  a6 : MATLAB Function  TreatAsAtomicUnit=on
  a7 : MATLAB Function  TreatAsAtomicUnit=on
  a8 : MATLAB Function  TreatAsAtomicUnit=on
  a9 : MATLAB Function  TreatAsAtomicUnit=on
  alpha1 : MATLAB Function  Commented=on  TreatAsAtomicUnit=on
  d23 : MATLAB Function  TreatAsAtomicUnit=on
  dL1 : MATLAB Function  TreatAsAtomicUnit=on
  dL2 : MATLAB Function  TreatAsAtomicUnit=on
  ddroux2 : MATLAB Function  TreatAsAtomicUnit=on
  ddrouy : MATLAB Function  TreatAsAtomicUnit=on
  dot,dji : MATLAB Function  TreatAsAtomicUnit=on
  dot,dji1 : MATLAB Function  TreatAsAtomicUnit=on
  dot,dji2 : MATLAB Function  TreatAsAtomicUnit=on
  dot,phiji : MATLAB Function  TreatAsAtomicUnit=on
  dot,phiji1 : MATLAB Function  TreatAsAtomicUnit=on
  dot,phiji2 : MATLAB Function  TreatAsAtomicUnit=on
  droux : MATLAB Function  TreatAsAtomicUnit=on
  drouy1 : MATLAB Function  TreatAsAtomicUnit=on
  phi23 : MATLAB Function  TreatAsAtomicUnit=on
  phiL1 : MATLAB Function  TreatAsAtomicUnit=on
  phiL2 : MATLAB Function  TreatAsAtomicUnit=on
  pi/1 : Integrator  Commented=on  InitialCondition=pi/7
  pi/6→pi/2 : Integrator  Commented=on  InitialCondition=pi/3
  pi/9 : Integrator  InitialCondition=pi/7
  roux1 : MATLAB Function  TreatAsAtomicUnit=on
  rouy1 : MATLAB Function  TreatAsAtomicUnit=on
  tauiL : Scope
  tauiR : Scope
  u1d : MATLAB Function  TreatAsAtomicUnit=on
  u1d1 : MATLAB Function  TreatAsAtomicUnit=on
  u1d2 : MATLAB Function  TreatAsAtomicUnit=on
  u1p : MATLAB Function  TreatAsAtomicUnit=on
  u1p1 : MATLAB Function  TreatAsAtomicUnit=on
  u1p2 : MATLAB Function  TreatAsAtomicUnit=on
  原常数 : Constant  Value=0.0000698
  原常数1 : Constant  Commented=on  Value=0.0000698
  原常数2 : Constant  Commented=on  Value=0.0000698
  试一下增大 : Constant  Commented=on  Value=10
  试一下增大1 : Constant  Commented=on  Value=10
  试一下增大2 : Constant  Commented=on  Value=10
  试一下增大3 : Constant  Commented=on  Value=100
  试一下增大4 : Constant  Commented=on  Value=100
  调大这个可以抑制突变，但是会增大输入绝对值 : Constant  Commented=on  Value=0.9
  调大这个可以抑制突变，但是会增大输入绝对值{1,4..7} (5 alike) : Constant  Commented=on  Value=1.5
  调大这个可以抑制突变，但是会增大输入绝对值10 : Constant  Commented=on  Value=0.1
  调大这个可以抑制突变，但是会增大输入绝对值11 : Constant  Value=0.1
  调大这个可以抑制突变，但是会增大输入绝对值{8..9,12..13} (4 alike) : Constant  Commented=on
  调大这个可以抑制突变，但是会增大输入绝对值2 : Constant  Commented=on  Value=0.9
  调大这个可以抑制突变，但是会增大输入绝对值3 : Constant  Commented=on  Value=0.9
  调大这个可以降低正输入，增大负输入 : Constant  Commented=on  Value=3000
  调大这个可以降低正输入，增大负输入{1,4..7} (5 alike) : Constant  Commented=on  Value=0.3
  调大这个可以降低正输入，增大负输入10 : Constant  Commented=on  Value=0.2
  调大这个可以降低正输入，增大负输入11 : Constant  Value=0.2
  调大这个可以降低正输入，增大负输入{8..9,12..13} (4 alike) : Constant  Commented=on  Value=0.0001
  调大这个可以降低正输入，增大负输入2 : Constant  Commented=on  Value=3000
  调大这个可以降低正输入，增大负输入3 : Constant  Commented=on  Value=3000
  越大phid超调越大 : Constant  Commented=on
  越大phid超调越大{1..3,5,7} (5 alike) : Constant  Commented=on  Value=0.5
  越大phid超调越大4 : Constant  Commented=on  Value=0.1
  越大phid超调越大6 : Constant  Value=0.5
  越大phid超调越大8 : Constant  Commented=on  Value=0.1
  越大phip超调越大 : Constant  Commented=on  Value=2.3
  越大phip超调越大{1..3,7} (4 alike) : Constant  Commented=on  Value=2.31
  越大phip超调越大4 : Constant  Commented=on  Value=0.4
  越大phip超调越大5 : Constant  Commented=on  Value=10
  越大phip超调越大6 : Constant  Value=10
  越大phip超调越大8 : Constant  Commented=on  Value=0.4
  tag scope: J=global, M=global, ddroud=global, ddroup=global, droud=global, droup=global, h=global, kroud=global, kroup=global, l=global, omg1=global, omg2=global, omg3=global, omgL=global, r=global, rd23=global, rdL1=global, rdL2=global, roud00=global, roud0=global, roud=global, roup00=global, roup0=global, roup=global, rphi23=global, rphiL1=global, rphiL2=global, theta1=global, theta2=global, theta3=global, thetaL=global, u1d=global, u1p=global, v1=global, v2=global, v3=global, vL=global, x1=global, x2=global, x3=global, xL=global, y1=global, y2=global, y3=global, yL=global
  wires:
  [omgL] -> dot,dji/5(omgj)
  dL1/1(y) -> Scope27/1, [dL1]
  [arfL1] -> dot,phiji/8(arfji)
  [y2] -> dL2/3(yi)
  [theta1] -> phiL1/5(thetai)
  Constant138/1 -> [rphiL2]
  dot,phiji/2(darfji) -> [darfL1]
  dot,phiji/1(dphiji) -> Mux28/1, [dphiL1]  "dphiL1"
  [thetaL] -> phiL1/6(thetaj)
  [v1] -> dot,phiji/3(vi)
  [u1d] -> MATLAB Function1/5(uid)
  [dL1] -> Add12/1
  [h] -> dot,phiji/5(h)
  [u1p] -> MATLAB Function1/6(uip)
  [y1] -> dL1/3(yi)
  [h] -> dot,dji/3(h)
  [omgL] -> dot,phiji/7(omgj)
  [x1] -> dL1/1(xi)
  phiL1/2(phiji) -> Scope39/1, [phiL1]
  [phiL1] -> Add14/1
  [dL1] -> dot,phiji/2(dji)
  phiL1/1(arfji) -> [arfL1], Scope24/1
  [yL] -> phiL1/3(yj)
  [arfL1] -> dot,dji/6(arfji)
  [vL] -> dot,phiji/6(vj)
  [xL] -> phiL1/1(xj)
  [omg1] -> dot,phiji/1(omgi)
  [v1] -> dot,dji/1(vi)
  [x1] -> phiL1/2(xi)
  [phiL1] -> dot,dji/2(phiji)
  [phiL1] -> dot,phiji/4(phiji)
  dot,dji/1(y) -> [ddL1]
  [y1] -> phiL1/4(yi)
  [yL] -> dL2/4(yj)
  [vL] -> dot,dji/7(vj)
  [x2] -> dL2/1(xi)
  dL2/1(y) -> [dL2]
  [yL] -> dL1/4(yj)
  [xL] -> dL1/2(xj)
  [rdL1] -> Add12/2
  MATLAB Function1/1(tauiL) -> Saturation10/1
  Constant133/1 -> [rphiL1]
  [xL] -> dL2/2(xj)
  [rphiL1] -> Add14/2
  Constant3/1 -> [rdL1]
  Add14/1 -> Scope3/1, Display28/1, [e1p]
  Add12/1 -> Display27/1, [e1d], Scope/1
  Constant4/1 -> [rdL2]
  [vL] -> dot,dji1/7(vj)
  dot,dji1/1(y) -> [ddL2]
  [phiL2] -> dot,dji1/2(phiji)
  [v2] -> dot,dji1/1(vi)
  [arfL2] -> dot,dji1/6(arfji)
  [omg2] -> dot,dji1/4(omgi)
  [h] -> dot,dji1/3(h)
  [omgL] -> dot,dji1/5(omgj)
  [y2] -> phiL2/4(yi)
  [x2] -> phiL2/2(xi)
  [xL] -> phiL2/1(xj)
  [yL] -> phiL2/3(yj)
  phiL2/1(arfji) -> Scope1/1, [arfL2]
  phiL2/2(phiji) -> Scope40/1, [phiL2]
  [thetaL] -> phiL2/6(thetaj)
  [theta2] -> phiL2/5(thetai)
  [phiL2] -> dot,phiji1/4(phiji)
  [omg2] -> dot,phiji1/1(omgi)
  [vL] -> dot,phiji1/6(vj)
  [dL2] -> dot,phiji1/2(dji)
  [omgL] -> dot,phiji1/7(omgj)
  [h] -> dot,phiji1/5(h)
  [v2] -> dot,phiji1/3(vi)
  dot,phiji1/2(darfji) -> [darfL2]
  [arfL2] -> dot,phiji1/8(arfji)
  Add1/1 -> [e2d], Scope2/1
  Add2/1 -> [e2p], Scope4/1
  [rphiL2] -> Add2/2
  [rdL2] -> Add1/2
  [phiL2] -> Add2/1
  [dL2] -> Add1/1
  [kroud] -> roux1/3(krou)
  [kroud] -> droux/1(krou)
  [roup0] -> drouy1/2(rou0)
  [roud00] -> droux/3(rou00)
  Constant48/1 -> [roup00]
  [roup00] -> rouy1/2(rou00)
  Clock3/1 -> drouy1/4(t)
  [roup0] -> rouy1/1(rou0)
  [kroup] -> drouy1/1(krou)
  Clock/1 -> roux1/4(t)
  [kroup] -> rouy1/3(krou)
  Constant33/1 -> [roud0]
  [roup00] -> drouy1/3(rou00)
  Clock1/1 -> droux/4(t)
  roux1/1(y) -> Scope11/1, [roud]
  [roud0] -> roux1/1(rou0)
  Constant28/1 -> [roud00]
  Constant47/1 -> [kroup]
  droux/1(y) -> Scope48/1, [droud]
  drouy1/1(y) -> [droup]
  Clock2/1 -> rouy1/4(t)
  Constant27/1 -> [kroud]
  [roud00] -> roux1/2(rou00)
  rouy1/1(y) -> Scope47/1, [roup]
  Constant49/1 -> [roup0]
  [roud0] -> droux/2(rou0)
  u1d/1(y) -> Display19/1, [u1d]
  [e1d] -> Mux48/2
  Product107/1 -> Mux50/1
  From613/1 -> Product107/1
  From617/1 -> Product106/2
  [k1roup] -> Gain1/1
  From615/1 -> Gain3/1
  From611/1 -> Product108/2
  [roud] -> Product95/2
  From612/1 -> Product106/3
  From506/1 -> Product105/3
  From610/1 -> Mux51/2
  Product105/1 -> Mux50/3
  [e1p] -> Mux49/2
  [k1roud] -> Gain/1
  Gain/1 -> Product95/1
  From616/1 -> Product108/1
  [roud] -> Mux48/1
  Gain3/1 -> Product106/1
  Gain1/1 -> Product96/1
  From504/1 -> Mux50/2
  Product96/1 -> Mux49/3
  Product106/1 -> Mux51/3
  From505/1 -> Product107/2
  Mux50/1 -> Scope51/1
  From614/1 -> Product105/2
  Mux49/1 -> Scope50/1
  Product95/1 -> Mux48/3
  Product108/1 -> Mux51/1
  [roup] -> Product96/2
  Mux51/1 -> Scope52/1
  Gain2/1 -> Product105/1
  [roup] -> Mux49/1
  From507/1 -> Gain2/1
  From221/1 -> Gain6/1
  [roup] -> Mux2/1
  Gain6/1 -> Product5/1
  Mux4/1 -> Scope13/1
  [roup] -> Product10/2
  Product8/1 -> Mux4/1
  Product9/1 -> Mux1/3
  Mux2/1 -> Scope10/1
  From226/1 -> Product5/2
  Mux1/1 -> Scope9/1
  Mux3/1 -> Scope12/1
  From219/1 -> Product7/2
  Product6/1 -> Mux4/3
  Product10/1 -> Mux2/3
  From218/1 -> Mux3/2
  Gain5/1 -> Product10/1
  Gain7/1 -> Product6/1
  [roud] -> Mux1/1
  From228/1 -> Product8/1
  Gain4/1 -> Product9/1
  [k2roud] -> Gain4/1
  [e2p] -> Mux2/2
  Product5/1 -> Mux3/3
  From222/1 -> Mux4/2
  From220/1 -> Product5/3
  From224/1 -> Product6/3
  [roud] -> Product9/2
  From223/1 -> Product8/2
  From227/1 -> Gain7/1
  [k2roup] -> Gain5/1
  From235/1 -> Product6/2
  From225/1 -> Product7/1
  Product7/1 -> Mux3/1
  [e2d] -> Mux1/2  "e2d"
  Constant31/1 -> [rd23]
  Constant32/1 -> ?
  [x2] -> d23/2(xj)
  d23/1(y) -> [d23]
  [x3] -> d23/1(xi)
  [y2] -> d23/4(yj)
  [y3] -> d23/3(yi)
  [omg2] -> dot,dji2/5(omgj)
  [h] -> dot,dji2/3(h)
  [omg3] -> dot,dji2/4(omgi)
  [arf23] -> dot,dji2/6(arfji)
  [v3] -> dot,dji2/1(vi)
  [phi23] -> dot,dji2/2(phiji)
  dot,dji2/1(y) -> [dd23]
  [v2] -> dot,dji2/7(vj)
  [theta3] -> phi23/5(thetai)
  [theta2] -> phi23/6(thetaj)
  phi23/2(phiji) -> Scope41/1, [phi23]
  phi23/1(arfji) -> [arf23], Scope14/1
  [y2] -> phi23/3(yj)
  [x2] -> phi23/1(xj)
  [x3] -> phi23/2(xi)
  [y3] -> phi23/4(yi)
  [arf23] -> dot,phiji2/8(arfji)
  dot,phiji2/2(darfji) -> [darf23]
  dot,phiji2/1(dphiji) -> Mux22/1, Mux28/3, [dphi23p]  "dphi23"
  [v3] -> dot,phiji2/3(vi)
  [h] -> dot,phiji2/5(h)
  [omg2] -> dot,phiji2/7(omgj)
  [d23] -> dot,phiji2/2(dji)
  [v2] -> dot,phiji2/6(vj)
  [omg3] -> dot,phiji2/1(omgi)
  [phi23] -> dot,phiji2/4(phiji)
  [e3d] -> Mux5/2
  Product14/1 -> Mux7/1
  From371/1 -> Product14/1
  From375/1 -> Product13/2
  [k3roup] -> Gain9/1
  From373/1 -> Gain11/1
  From369/1 -> Product15/2
  [roud] -> Product16/2
  From370/1 -> Product13/3
  From366/1 -> Product12/3
  From368/1 -> Mux8/2
  Product12/1 -> Mux7/3
  [e3p] -> Mux6/2
  [k3roud] -> Gain8/1
  Gain8/1 -> Product16/1
  From374/1 -> Product15/1
  [roud] -> Mux5/1
  Gain11/1 -> Product13/1
  Gain9/1 -> Product11/1
  From364/1 -> Mux7/2
  Product11/1 -> Mux6/3
  Product13/1 -> Mux8/3
  From365/1 -> Product14/2
  Mux7/1 -> Scope18/1
  Mux5/1 -> Scope25/1
  From372/1 -> Product12/2
  Mux6/1 -> Scope17/1
  Product16/1 -> Mux5/3
  Product15/1 -> Mux8/1
  [roup] -> Product11/2
  Mux8/1 -> Scope19/1
  Gain10/1 -> Product12/1
  [roup] -> Mux6/1
  From367/1 -> Gain10/1
  [d23] -> Add3/1
  [phi23] -> Add4/1
  [rd23] -> Add3/2
  [rphi23] -> Add4/2
  Add4/1 -> Scope28/1, [e3p]
  Add3/1 -> Scope26/1, [e3d]
  [rphiL2] -> MATLAB Function18/1(rphiL2)
  [theta2] -> Scope29/1, MATLAB Function18/3(theta2)
  [thetaL] -> Scope30/1, MATLAB Function18/2(thetaL)
  [dphi23p] -> Add/1
  [omgL] -> Add/2
  [omg2] -> Add/3
  Add/1 -> Mux22/2, [dphi23]  "dphi23"
  [xL] -> MATLAB Function30/7(xL)
  Mux63/1 -> Scope31/1, To Workspace13/1
  MATLAB Function30/3(JI2) -> Scope102/1, Mux78/3
  MATLAB Function30/4(JI3) -> Scope103/1, Mux78/4
  MATLAB Function30/7(yier) -> Scope106/1
  [x3] -> MATLAB Function30/5(x3)
  [y2] -> MATLAB Function30/4(y2)
  MATLAB Function30/5(yil) -> Mux63/1, Scope104/1  "1L"
  MATLAB Function30/8(saner) -> Mux63/4, Scope107/1  "32"
  MATLAB Function30/2(JI1) -> Scope101/1, Mux78/2
  MATLAB Function30/6(sanyi) -> Mux63/2, Scope105/1  "31"
  MATLAB Function30/1(JIL) -> Scope100/1, Mux78/1
  [x2] -> MATLAB Function30/3(x2)
  [x1] -> MATLAB Function30/1(x1)
  [y3] -> MATLAB Function30/6(y3)
  [yL] -> MATLAB Function30/8(yL)
  MATLAB Function30/9(erl) -> Scope108/1, Mux63/3  "21"
  Mux78/1 -> Scope32/1, To Workspace15/1
  [y1] -> MATLAB Function30/2(y1)
  From399/1 -> Gain14/1
  [roup] -> [eupp], Mux10/1  "up bound"
  Gain14/1 -> Product17/1
  Mux12/1 -> Scope36/1
  [roup] -> Product22/2
  Product20/1 -> Goto108/1, Mux12/1  "up bound"
  Product21/1 -> [edod], Mux9/5  "low bound"
  Mux10/1 -> To Workspace9/1, Scope34/1
  From404/1 -> Product17/2
  Mux9/1 -> To Workspace/1, Scope33/1
  Mux11/1 -> Scope35/1
  From397/1 -> Product19/2
  Product18/1 -> Goto109/1, Mux12/5  "low bound"
  Product22/1 -> [edop], Mux10/5  "low bound"
  From396/1 -> Mux11/2  "S1d"
  Gain13/1 -> Product22/1
  Gain15/1 -> Product18/1
  [roud] -> [eupd], Mux9/1  "up bound"
  From406/1 -> Product20/1
  Gain12/1 -> Product21/1
  [ked] -> Gain12/1
  [e1p] -> Mux10/2  "E1p"
  Product17/1 -> Goto107/1, Mux11/5  "low bound"
  From400/1 -> Mux12/2  "S1p"
  From398/1 -> Product17/3
  From402/1 -> Product18/3
  [roud] -> Product21/2
  From401/1 -> Product20/2
  From405/1 -> Gain15/1
  [kep] -> Gain13/1
  From407/1 -> Product18/2
  From403/1 -> Product19/1
  Product19/1 -> Goto106/1, Mux11/1  "up bound"
  [e1d] -> Mux9/2  "E1d"
  From408/1 -> Mux11/3  "S2d"
  From415/1 -> Mux11/4  "S3d"
  From417/1 -> Mux12/4  "S3P"
  From416/1 -> Mux12/3  "S2P"
  [e3d] -> Mux9/4  "E3d"
  [e2d] -> Mux9/3  "E2d"
  [e2p] -> Mux10/3  "E2p"
  [e3p] -> Mux10/4  "E3p"
  From741/1 -> Mux17/32
  Mux17/1 -> To Workspace49/1
  From713/1 -> Mux17/11
  From716/1 -> Mux17/9
  From712/1 -> Mux17/10
  From718/1 -> Mux17/23
  From721/1 -> Mux17/19
  From709/1 -> Mux17/14
  From723/1 -> Mux17/17
  From714/1 -> Mux17/7
  From711/1 -> Mux17/16
  From740/1 -> Mux17/28
  From710/1 -> Mux17/15
  From726/1 -> Mux17/26
  From722/1 -> Mux17/18
  From705/1 -> Mux17/5
  From725/1 -> Mux17/21
  From717/1 -> Mux17/22
  From706/1 -> Mux17/6
  From707/1 -> Mux17/12
  From703/1 -> Mux17/3
  From715/1 -> Mux17/8
  From733/1 -> Mux17/35
  From719/1 -> Mux17/24
  From708/1 -> Mux17/13
  From729/1 -> Mux17/34
  Clock19/1 -> Mux17/1
  From732/1 -> Mux17/30
  From742/1 -> Mux17/33
  From704/1 -> Mux17/4
  From736/1 -> Mux17/31
  From683/1 -> Mux17/2
  From727/1 -> Mux17/27
  From728/1 -> Mux17/29
  From720/1 -> Mux17/25
  From724/1 -> Mux17/20
  MATLAB Function12/2(domg1) -> [domg1], Scope82/1
  Constant144/1 -> [M]
  Constant146/1 -> [l]
  MATLAB Function12/1(dv1) -> [dv1], Display41/1, Scope81/1
  Constant145/1 -> [r]
  Constant147/1 -> [J]
  From743/1 -> Mux17/37
  From737/1 -> Mux17/36
  From744/1 -> Mux17/38
  From730/1 -> Mux17/39
  From734/1 -> Mux17/40
  From774/1 -> Mux17/41
  From745/1 -> Mux17/42
  From746/1 -> Mux17/43
  From731/1 -> Mux17/44
  From735/1 -> Mux17/45
  From739/1 -> Mux17/46
  From747/1 -> Mux17/47
  [roud] -> Divide/2
  [e1d] -> Divide/1
  Divide/1 -> [z1d]
  Divide1/1 -> [z1p]
  [e1p] -> Divide1/1
  [roud] -> Divide1/2
  [roud] -> Divide3/2
  [e2p] -> Divide3/1
  Divide3/1 -> [z2p]
  Divide2/1 -> [z2d]
  [e2d] -> Divide2/1
  [roud] -> Divide2/2
  [roud] -> Divide4/2
  [e3d] -> Divide4/1
  Divide4/1 -> [z3d]
  Divide5/1 -> [z3p]
  [e3p] -> Divide5/1
  [roud] -> Divide5/2
  Constant46/1 -> [upz1d]
  Constant50/1 -> [upz2d]
  Constant51/1 -> [upz3d]
  Constant54/1 -> [upz3p]
  Constant53/1 -> [upz2p]
  Constant52/1 -> [upz1p]
  Fcn/1 -> [lowz1d]
  Mux/1 -> Fcn/1
  [roud0] -> Mux/1
  [roud00] -> Mux/2
  [rdL1] -> Mux/3
  [rdL2] -> Mux13/3
  [roud00] -> Mux13/2
  [roud0] -> Mux13/1
  Mux13/1 -> Fcn1/1
  Fcn1/1 -> [lowz2d]
  Fcn2/1 -> [lowz3d]
  Mux14/1 -> Fcn2/1
  [roud0] -> Mux14/1
  [roud00] -> Mux14/2
  [rd23] -> Mux14/3
  [rphiL1] -> Mux15/2
  [roup0] -> Mux15/1
  Mux15/1 -> Fcn3/1
  Fcn3/1 -> Scope70/1, [lowz1p]
  Fcn4/1 -> Scope68/1, [lowz2p]
  Mux16/1 -> Fcn4/1
  [roup0] -> Mux16/1
  [rphiL2] -> Mux16/2
  [rphi23] -> Mux18/2
  [roup0] -> Mux18/1
  Mux18/1 -> Fcn5/1
  [omg1] -> MATLAB Function7/4(wi)
  [omgL] -> MATLAB Function7/3(wj)
  [vL] -> MATLAB Function7/1(vj)
  [v1] -> MATLAB Function7/2(vi)
  [arfL1] -> MATLAB Function7/6(a)
  [phiL1] -> MATLAB Function7/5(phi)
  [h] -> MATLAB Function7/7(h)
  MATLAB Function7/1(doted) -> [de1d]
  MATLAB Function8/1(doted) -> [de2d]
  [h] -> MATLAB Function8/7(h)
  [phiL2] -> MATLAB Function8/5(phi)
  [arfL2] -> MATLAB Function8/6(a)
  [v2] -> MATLAB Function8/2(vi)
  [vL] -> MATLAB Function8/1(vj)
  [omgL] -> MATLAB Function8/3(wj)
  [omg2] -> MATLAB Function8/4(wi)
  [omg3] -> MATLAB Function10/4(wi)
  [omg2] -> MATLAB Function10/3(wj)
  [v2] -> MATLAB Function10/1(vj)
  [v3] -> MATLAB Function10/2(vi)
  [arf23] -> MATLAB Function10/6(a)
  [phi23] -> MATLAB Function10/5(phi)
  [h] -> MATLAB Function10/7(h)
  MATLAB Function10/1(doted) -> [de3d]
  MATLAB Function13/1(dotep) -> [de1p]
  [h] -> MATLAB Function13/7(h)
  [phiL1] -> MATLAB Function13/5(phi)
  [arfL1] -> MATLAB Function13/6(a)
  [v1] -> MATLAB Function13/2(vi)
  [vL] -> MATLAB Function13/1(vj)
  [omgL] -> MATLAB Function13/3(wj)
  [omg1] -> MATLAB Function13/4(wi)
  [dL1] -> MATLAB Function13/8(d)
  [dL2] -> MATLAB Function11/8(d)
  [omg2] -> MATLAB Function11/4(wi)
  [omgL] -> MATLAB Function11/3(wj)
  [vL] -> MATLAB Function11/1(vj)
  [v2] -> MATLAB Function11/2(vi)
  [arfL2] -> MATLAB Function11/6(a)
  [phiL2] -> MATLAB Function11/5(phi)
  [h] -> MATLAB Function11/7(h)
  MATLAB Function11/1(dotep) -> [de2p]
  MATLAB Function14/1(dotep) -> [de3p]
  [h] -> MATLAB Function14/7(h)
  [phi23] -> MATLAB Function14/5(phi)
  [arf23] -> MATLAB Function14/6(a)
  [v3] -> MATLAB Function14/2(vi)
  [v2] -> MATLAB Function14/1(vj)
  [omg2] -> MATLAB Function14/3(wj)
  [omg3] -> MATLAB Function14/4(wi)
  [d23] -> MATLAB Function14/8(d)
  [roud0] -> ddroux2/2(rou0)
  ddroux2/1(y) -> [ddroud], Scope42/1
  Clock6/1 -> ddroux2/4(t)
  [roud00] -> ddroux2/3(rou00)
  [kroud] -> ddroux2/1(krou)
  ddrouy/1(y) -> [ddroup]
  [roup00] -> ddrouy/3(rou00)
  [kroup] -> ddrouy/1(krou)
  Clock7/1 -> ddrouy/4(t)
  [roup0] -> ddrouy/2(rou0)
  [vL] -> MATLAB Function15/1(vj)
  [v1] -> MATLAB Function15/2(vi)
  [omgL] -> MATLAB Function15/3(wj)
  [omg1] -> MATLAB Function15/4(wi)
  [arfL1] -> MATLAB Function15/5(a)
  [phiL1] -> MATLAB Function15/6(phi)
  [h] -> MATLAB Function15/7(h)
  [e1d] -> MATLAB Function15/8(ed)
  [roud] -> MATLAB Function15/9(roud)
  [z1d] -> MATLAB Function15/11(zd)
  [upz1d] -> MATLAB Function15/12(upzd)
  [lowz1d] -> MATLAB Function15/13(lowzd)
  [k1d] -> MATLAB Function15/14(kd)
  MATLAB Function15/1(delta1) -> [delta11]
  [droud] -> MATLAB Function15/10(droud)
  [phiL1] -> MATLAB Function19/6(phi)
  [droup] -> MATLAB Function19/10(droup)
  [arfL1] -> MATLAB Function19/5(a)
  [h] -> MATLAB Function19/7(h)
  [k1p] -> MATLAB Function19/14(kp)
  [lowz1p] -> MATLAB Function19/13(lowzp)
  [omg1] -> MATLAB Function19/4(wi)
  [upz1p] -> MATLAB Function19/12(upzp)
  [omgL] -> MATLAB Function19/3(wj)
  [z1p] -> MATLAB Function19/11(zp)
  [e1p] -> MATLAB Function19/8(ep)
  [roup] -> MATLAB Function19/9(roup)
  [vL] -> MATLAB Function19/1(vj)
  [v1] -> MATLAB Function19/2(vi)
  [dL1] -> MATLAB Function19/15(d)
  MATLAB Function19/1(delta2) -> [delta12]
  MATLAB Function21/1(delta2) -> [delta22]
  [dL2] -> MATLAB Function21/15(d)
  [v2] -> MATLAB Function21/2(vi)
  [vL] -> MATLAB Function21/1(vj)
  [roup] -> MATLAB Function21/9(roup)
  [e2p] -> MATLAB Function21/8(ep)
  [z2p] -> MATLAB Function21/11(zp)
  [omgL] -> MATLAB Function21/3(wj)
  [upz2p] -> MATLAB Function21/12(upzp)
  [omg2] -> MATLAB Function21/4(wi)
  [lowz2p] -> MATLAB Function21/13(lowzp)
  [k2p] -> MATLAB Function21/14(kp)
  [h] -> MATLAB Function21/7(h)
  [arfL2] -> MATLAB Function21/5(a)
  [droup] -> MATLAB Function21/10(droup)
  [phiL2] -> MATLAB Function21/6(phi)
  [droud] -> MATLAB Function20/10(droud)
  MATLAB Function20/1(delta1) -> [delta21]
  [k2d] -> MATLAB Function20/14(kd)
  [lowz2d] -> MATLAB Function20/13(lowzd)
  [upz2d] -> MATLAB Function20/12(upzd)
  [z2d] -> MATLAB Function20/11(zd)
  [roud] -> MATLAB Function20/9(roud)
  [e2d] -> MATLAB Function20/8(ed)
  [h] -> MATLAB Function20/7(h)
  [phiL2] -> MATLAB Function20/6(phi)
  [arfL2] -> MATLAB Function20/5(a)
  [omg2] -> MATLAB Function20/4(wi)
  [omgL] -> MATLAB Function20/3(wj)
  [v2] -> MATLAB Function20/2(vi)
  [vL] -> MATLAB Function20/1(vj)
  [v2] -> MATLAB Function22/1(vj)
  [v3] -> MATLAB Function22/2(vi)
  [omg2] -> MATLAB Function22/3(wj)
  [omg3] -> MATLAB Function22/4(wi)
  [arf23] -> MATLAB Function22/5(a)
  [phi23] -> MATLAB Function22/6(phi)
  [h] -> MATLAB Function22/7(h)
  [e3d] -> MATLAB Function22/8(ed)
  [roud] -> MATLAB Function22/9(roud)
  [z3d] -> MATLAB Function22/11(zd)
  [upz3d] -> MATLAB Function22/12(upzd)
  [lowz3d] -> MATLAB Function22/13(lowzd)
  [k3d] -> MATLAB Function22/14(kd)
  MATLAB Function22/1(delta1) -> [delta31]
  [droud] -> MATLAB Function22/10(droud)
  [phi23] -> MATLAB Function23/6(phi)
  [droup] -> MATLAB Function23/10(droup)
  [arf23] -> MATLAB Function23/5(a)
  [h] -> MATLAB Function23/7(h)
  [k3p] -> MATLAB Function23/14(kp)
  [lowz3p] -> MATLAB Function23/13(lowzp)
  [omg3] -> MATLAB Function23/4(wi)
  [upz3p] -> MATLAB Function23/12(upzp)
  [omg2] -> MATLAB Function23/3(wj)
  [z3p] -> MATLAB Function23/11(zp)
  [e3p] -> MATLAB Function23/8(ep)
  [roup] -> MATLAB Function23/9(roup)
  [v2] -> MATLAB Function23/1(vj)
  [v3] -> MATLAB Function23/2(vi)
  [d23] -> MATLAB Function23/15(d)
  MATLAB Function23/1(delta2) -> [delta32]
  [vL] -> u1d/1(vj)
  [omgL] -> u1d/3(wj)
  [v1] -> Mux27/1, u1d/2(vi)
  [omg1] -> Mux27/2, u1d/4(wi)
  [e1d] -> u1d/6(eid)
  [de1d] -> u1d/7(doteid)
  [roud] -> u1d/8(roud)
  [ddroud] -> u1d/10(ddotroud)
  [droud] -> u1d/9(dotroud)
  [z1d] -> u1d/11(zid)
  [upz1d] -> u1d/13(upzid)
  [lowz1d] -> u1d/14(lowzid)
  [phiL1] -> u1d/15(phi)
  [dphiL1] -> u1d/16(dotphi)
  [arfL1] -> u1d/17(a)
  [darfL1] -> u1d/18(dota)
  [k1d] -> u1d/19(kid)
  [h] -> u1d/20(h)
  [D1dm_hat] -> u1d/21(Didm)
  [k1ed] -> u1d/22(kied)
  [dotz1d] -> u1d/12(dotzid)
  MATLAB Function24/1(y) -> [dotz1d]
  [e1d] -> MATLAB Function24/1(eid)
  [de1d] -> MATLAB Function24/2(doteid)
  [roud] -> MATLAB Function24/3(roud)
  [droud] -> MATLAB Function24/4(dotroud)
  [droud] -> MATLAB Function25/4(dotroud)
  [roud] -> MATLAB Function25/3(roud)
  [de2d] -> MATLAB Function25/2(doteid)
  [e2d] -> MATLAB Function25/1(eid)
  MATLAB Function25/1(y) -> [dotz2d]
  MATLAB Function26/1(y) -> [dotz3d]
  [e3d] -> MATLAB Function26/1(eid)
  [de3d] -> MATLAB Function26/2(doteid)
  [roud] -> MATLAB Function26/3(roud)
  [droud] -> MATLAB Function26/4(dotroud)
  [droup] -> MATLAB Function27/4(dotroup)
  [roup] -> MATLAB Function27/3(roup)
  [de1p] -> MATLAB Function27/2(doteip)
  [e1p] -> MATLAB Function27/1(eip)
  MATLAB Function27/1(y) -> [dotz1p]
  MATLAB Function28/1(y) -> [dotz2p]
  [e2p] -> MATLAB Function28/1(eip)
  [de2p] -> MATLAB Function28/2(doteip)
  [roup] -> MATLAB Function28/3(roup)
  [droup] -> MATLAB Function28/4(dotroup)
  [droup] -> MATLAB Function29/4(dotroup)
  [roup] -> MATLAB Function29/3(roup)
  [de3p] -> MATLAB Function29/2(doteip)
  [e3p] -> MATLAB Function29/1(eip)
  MATLAB Function29/1(y) -> [dotz3p]
  [dotz1p] -> u1p/12(dotzip)
  [k1ep] -> u1p/22(kiep)
  [D1pm_hat] -> u1p/21(Dipm)
  [h] -> u1p/20(h)
  [k1p] -> u1p/19(kip)
  [darfL1] -> u1p/18(dota)
  [arfL1] -> u1p/17(a)
  [dphiL1] -> u1p/16(dotphi)
  [phiL1] -> u1p/15(phi)
  [lowz1p] -> u1p/14(lowzip)
  [upz1p] -> u1p/13(upzip)
  [z1p] -> u1p/11(zip)
  [droup] -> u1p/9(dotroup)
  [ddroup] -> u1p/10(ddotroup)
  [roup] -> u1p/8(roup)
  [de1p] -> u1p/7(doteip)
  [e1p] -> u1p/6(eip)
  [omg1] -> u1p/4(wi)
  [v1] -> u1p/2(vi)
  [omgL] -> u1p/3(wj)
  [vL] -> u1p/1(vj)
  u1p/1(y) -> Display18/1, [u1p]
  [dL1] -> u1p/23(d)
  [ddL1] -> u1p/24(dotd)
  Constant/1 -> [h]
  [arfL1] -> a/1(a)
  [l] -> a/3(l)
  [J] -> a/4(j)
  [h] -> a/2(h)
  [r] -> a/5(r)
  [M] -> a/6(m)
  a/1(y) -> Display12/1, [aa]
  a1/1(y) -> Display13/1, [bb]
  [M] -> a1/6(m)
  [r] -> a1/5(r)
  [h] -> a1/2(h)
  [J] -> a1/4(j)
  [l] -> a1/3(l)
  [arfL1] -> a1/1(a)
  a2/1(y) -> Display14/1, [dd]
  [M] -> a2/6(m)
  [r] -> a2/5(r)
  [h] -> a2/2(h)
  [J] -> a2/4(j)
  [l] -> a2/3(l)
  [arfL1] -> a2/1(a)
  a3/1(y) -> Display15/1, [cc]
  [M] -> a3/6(m)
  [r] -> a3/5(r)
  [h] -> a3/2(h)
  [J] -> a3/4(j)
  [l] -> a3/3(l)
  [arfL1] -> a3/1(a)
  [dd] -> MATLAB Function1/4(dd)
  [cc] -> MATLAB Function1/3(cc)
  [bb] -> MATLAB Function1/2(bb)
  [aa] -> MATLAB Function1/1(aa)
  [aa] -> MATLAB Function2/1(aa)
  [bb] -> MATLAB Function2/2(bb)
  [cc] -> MATLAB Function2/3(cc)
  [dd] -> MATLAB Function2/4(dd)
  MATLAB Function2/1(tauiR) -> Saturation11/1
  [u1p] -> MATLAB Function2/6(uip)
  [u1d] -> MATLAB Function2/5(uid)
  [M] -> MATLAB Function12/5(m)
  [l] -> MATLAB Function12/6(l)
  [J] -> MATLAB Function12/4(J)
  [r] -> MATLAB Function12/3(r)
  [tau1R] -> MATLAB Function12/2(tauiR)
  [tau1L] -> MATLAB Function12/1(tauiL)
  Constant7/1 -> Goto52/1
  Constant17/1 -> Goto55/1
  Constant18/1 -> Goto180/1
  Constant19/1 -> Goto179/1
  Constant21/1 -> Goto175/1
  Constant20/1 -> Goto190/1
  Constant22/1 -> Goto173/1
  Constant23/1 -> Goto172/1
  Constant29/1 -> Goto170/1
  Constant26/1 -> Goto171/1
  Constant25/1 -> Goto133/1
  调大这个可以抑制突变，但是会增大输入绝对值/1 -> Goto134/1
  [omg1] -> dot,dji/4(omgi)
  Mux48/1 -> Scope49/1
  Mux20/1 -> Scope43/1
  [delta21] -> u1d1/5(deltaid)
  [delta22] -> u1p1/5(deltaip)
  [u2d] -> MATLAB Function32/5(uid)
  [u2p] -> MATLAB Function32/6(uip)
  MATLAB Function32/1(tauiR) -> Saturation9/1
  [aa2] -> MATLAB Function31/1(aa)
  [bb2] -> MATLAB Function31/2(bb)
  [cc2] -> MATLAB Function31/3(cc)
  [dd2] -> MATLAB Function31/4(dd)
  [ddL2] -> u1p1/24(dotd)
  [dL2] -> u1p1/23(d)
  u1p1/1(y) -> [u2p], Display26/1
  [vL] -> u1p1/1(vj)
  [omgL] -> u1p1/3(wj)
  [v2] -> u1p1/2(vi)
  [omg2] -> u1p1/4(wi)
  [e2p] -> u1p1/6(eip)
  [de2p] -> u1p1/7(doteip)
  [roup] -> u1p1/8(roup)
  [ddroup] -> u1p1/10(ddotroup)
  [droup] -> u1p1/9(dotroup)
  [z2p] -> u1p1/11(zip)
  [upz2p] -> u1p1/13(upzip)
  [lowz2p] -> u1p1/14(lowzip)
  [phiL2] -> u1p1/15(phi)
  [dphiL2] -> u1p1/16(dotphi)
  [arfL2] -> u1p1/17(a)
  [darfL2] -> u1p1/18(dota)
  [k2p] -> u1p1/19(kip)
  [h] -> u1p1/20(h)
  [D2pm_hat] -> u1p1/21(Dipm)
  [k2ep] -> u1p1/22(kiep)
  [dotz2p] -> u1p1/12(dotzip)
  [dotz2d] -> u1d1/12(dotzid)
  [k2ed] -> u1d1/22(kied)
  [D2dm_hat] -> u1d1/21(Didm)
  [h] -> u1d1/20(h)
  [k2d] -> u1d1/19(kid)
  [darfL2] -> u1d1/18(dota)
  [arfL2] -> u1d1/17(a)
  [dphiL2] -> u1d1/16(dotphi)
  [phiL2] -> u1d1/15(phi)
  [lowz2d] -> u1d1/14(lowzid)
  [upz2d] -> u1d1/13(upzid)
  [z2d] -> u1d1/11(zid)
  [droud] -> u1d1/9(dotroud)
  [ddroud] -> u1d1/10(ddotroud)
  [roud] -> u1d1/8(roud)
  [de2d] -> u1d1/7(doteid)
  [e2d] -> u1d1/6(eid)
  [omg2] -> u1d1/4(wi)
  [v2] -> u1d1/2(vi)
  [omgL] -> u1d1/3(wj)
  [vL] -> u1d1/1(vj)
  u1d1/1(y) -> Display29/1, [u2d]
  MATLAB Function31/1(tauiL) -> Saturation8/1, Display24/1
  [u2p] -> MATLAB Function31/6(uip)
  [u2d] -> MATLAB Function31/5(uid)
  [tau2L] -> MATLAB Function3/1(tauiL)
  [tau2R] -> MATLAB Function3/2(tauiR)
  [r] -> MATLAB Function3/3(r)
  [J] -> MATLAB Function3/4(J)
  [l] -> MATLAB Function3/6(l)
  [M] -> MATLAB Function3/5(m)
  MATLAB Function3/1(dv1) -> Scope45/1, [dv2]  "dv2"
  MATLAB Function3/2(domg1) -> Scope46/1, [domg2]  "domg2"
  调大这个可以降低正输入，增大负输入/1 -> Goto189/1
  Constant30/1 -> Goto174/1
  Constant36/1 -> Goto178/1
  Constant37/1 -> Goto177/1
  Constant38/1 -> Goto54/1
  Constant39/1 -> Goto51/1
  MATLAB Function4/2(domg1) -> [domg3], Scope54/1
  MATLAB Function4/1(dv1) -> [dv3], Scope53/1
  [M] -> MATLAB Function4/5(m)
  [l] -> MATLAB Function4/6(l)
  [J] -> MATLAB Function4/4(J)
  [r] -> MATLAB Function4/3(r)
  [tau3R] -> MATLAB Function4/2(tauiR)
  [tau3L] -> MATLAB Function4/1(tauiL)
  [u3d] -> MATLAB Function5/5(uid)
  [u3p] -> MATLAB Function5/6(uip)
  u1d2/1(y) -> [u3d], Display23/1
  [v2] -> Mux23/1, u1d2/1(vj)
  [omg2] -> Mux23/2, u1d2/3(wj)
  [v3] -> u1d2/2(vi)
  [omg3] -> u1d2/4(wi)
  [e3d] -> u1d2/6(eid)
  [de3d] -> u1d2/7(doteid)
  [roud] -> u1d2/8(roud)
  [ddroud] -> u1d2/10(ddotroud)
  [droud] -> u1d2/9(dotroud)
  [z3d] -> u1d2/11(zid)
  [upz3d] -> u1d2/13(upzid)
  [lowz3d] -> u1d2/14(lowzid)
  [phi23] -> u1d2/15(phi)
  [dphi23] -> u1d2/16(dotphi)
  [arf23] -> u1d2/17(a)
  [darf23] -> u1d2/18(dota)
  [k3d] -> u1d2/19(kid)
  [h] -> u1d2/20(h)
  [D3dm_hat] -> u1d2/21(Didm)
  [k3ed] -> u1d2/22(kied)
  [dotz3d] -> u1d2/12(dotzid)
  [dotz3p] -> u1p2/12(dotzip)
  [k3ep] -> u1p2/22(kiep)
  [D3pm_hat] -> u1p2/21(Dipm)
  [h] -> u1p2/20(h)
  [k3p] -> u1p2/19(kip)
  [darf23] -> u1p2/18(dota)
  [arf23] -> u1p2/17(a)
  [dphi23] -> u1p2/16(dotphi)
  [phi23] -> u1p2/15(phi)
  [lowz3p] -> u1p2/14(lowzip)
  [upz3p] -> u1p2/13(upzip)
  [z3p] -> u1p2/11(zip)
  [droup] -> u1p2/9(dotroup)
  [ddroup] -> u1p2/10(ddotroup)
  [roup] -> u1p2/8(roup)
  [de3p] -> u1p2/7(doteip)
  [e3p] -> u1p2/6(eip)
  [omg3] -> u1p2/4(wi)
  [v3] -> u1p2/2(vi)
  [omg2] -> u1p2/3(wj)
  [v2] -> u1p2/1(vj)
  u1p2/1(y) -> Display22/1, [u3p]
  [d23] -> u1p2/23(d)
  [dd23] -> u1p2/24(dotd)
  [dd3] -> MATLAB Function5/4(dd)
  [cc3] -> MATLAB Function5/3(cc)
  [bb3] -> MATLAB Function5/2(bb)
  [aa3] -> MATLAB Function5/1(aa)
  [u3p] -> MATLAB Function6/6(uip)
  [u3d] -> MATLAB Function6/5(uid)
  [delta32] -> u1p2/5(deltaip)
  [delta31] -> u1d2/5(deltaid)
  Mux21/1 -> Scope55/1
  Constant41/1 -> Goto53/1
  Constant40/1 -> Goto56/1
  试一下增大/1 -> Goto182/1
  Constant45/1 -> Goto181/1
  Constant56/1 -> Goto176/1
  Constant55/1 -> Goto191/1
  Mux22/1 -> Scope56/1
  From841/1 -> Cos18/1
  Cos15/1 -> Product43/2
  From857/1 -> Integrator31/1
  Integrator43/1 -> Display32/1, Goto225/1, To Workspace24/1
  From847/1 -> Sin24/1
  Sin21/1 -> Product44/3
  Integrator41/1 -> Product53/1, Goto222/1
  From831/1 -> Cos16/1
  Cos14/1 -> Product42/2
  Integrator33/1 -> Goto234/1, Product50/1
  From853/1 -> Product39/2
  Product46/1 -> Add24/1
  Integrator34/1 -> Goto233/1, To Workspace22/1
  Product41/1 -> Add22/2
  Cos16/1 -> Product46/2
  From840/1 -> Sin23/1
  Add22/1 -> Integrator43/1
  From462角速度1/1 -> Product52/1
  From345/1 -> Display31/1, Integrator42/1
  Add19/1 -> Integrator36/1
  From843/1 -> Integrator38/1
  From350/1 -> Product40/1
  Product51/1 -> Add19/1
  Integrator29/1 -> Goto229/1, To Workspace20/1
  From352/1 -> Sin19/1
  From842/1 -> Cos11/1
  Sin24/1 -> Product52/3
  From349/1 -> Product43/1
  From824/1 -> Integrator30/1
  From355/1 -> Integrator28/1
  From346/1 -> Display30/1, Integrator49/1
  Integrator40/1 -> Goto239/1
  Product42/1 -> Add22/1
  Product53/1 -> Add20/1
  Integrator31/1 -> Goto224/1
  Add20/1 -> Integrator45/1
  Product54/1 -> Add21/1
  Product40/1 -> Add23/2
  Integrator38/1 -> Goto237/1
  From353/1 -> Cos14/1
  From348/1 -> Sin18/1
  Product39/1 -> Add21/2
  Integrator26/1 -> Goto223/1, To Workspace19/1
  Integrator45/1 -> Goto221/1, To Workspace18/1
  Product52/1 -> Add20/2
  Cos13/1 -> Product54/2
  From854/1 -> Sin17/1
  Add21/1 -> Integrator26/1
  From835/1 -> Product49/2
  From855/1 -> Cos12/1
  Integrator35/1 -> Product49/1, Goto235/1
  Integrator27/1 -> To Workspace25/1, Goto228/1
  From836/1 -> Sin22/1
  From838/1 -> Product48/1
  Product44/1 -> Add17/2
  Sin23/1 -> Product48/3
  From851/1 -> Product54/1
  Integrator30/1 -> Mux24/2, Goto231/1, Product45/1  "omg2"
  Sin19/1 -> Product40/3
  Cos17/1 -> Product47/2
  Product49/1 -> Add18/2
  Cos18/1 -> Product50/2
  Add23/1 -> Integrator27/1
  From837/1 -> Product51/1
  Sin17/1 -> Product39/3
  Add24/1 -> Integrator29/1
  From856/1 -> Cos13/1
  Sin18/1 -> Product41/3
  From833/1 -> Integrator33/1
  Sin20/1 -> Product45/3
  From828/1 -> Product44/1
  Product45/1 -> Add24/2
  From827/1 -> Product47/1
  From846/1 -> Integrator40/1
  From829/1 -> Product44/2
  From347/1 -> Product41/2
  Add18/1 -> Integrator34/1
  From839/1 -> Product48/2
  From354/1 -> Cos15/1
  From852/1 -> Product39/1
  From834/1 -> Integrator35/1
  From845/1 -> Integrator39/1
  From830/1 -> Sin21/1
  From826/1 -> Sin20/1
  Product43/1 -> Add23/1
  Integrator39/1 -> Goto238/1
  Integrator36/1 -> Goto236/1, To Workspace23/1
  Add17/1 -> Integrator32/1
  Sin22/1 -> Product49/3
  From344/1 -> Integrator41/1
  Integrator28/1 -> Product46/1, Mux24/1, Goto230/1  "v2"
  From832/1 -> Cos17/1
  From844/1 -> Product52/2
  Product48/1 -> Add19/2
  Integrator32/1 -> Goto232/1, To Workspace21/1
  Cos12/1 -> Product53/2
  Product47/1 -> Add17/1
  From351/1 -> Product40/2
  Cos11/1 -> Product51/2
  From825/1 -> Product45/2
  Product50/1 -> Add18/1
  Mux23/1 -> Scope58/1
  Mux24/1 -> Scope57/1
  Integrator42/1 -> Mux25/1, Goto226/1, Product42/1  "v1"
  Integrator49/1 -> Mux25/2, Goto227/1, Product41/1  "omg1"
  Mux25/1 -> Scope59/1
  Mux27/1 -> Scope60/1
  dot,phiji1/1(dphiji) -> Mux28/2, [dphiL2]  "dphiL2"
  Mux28/1 -> Scope61/1
  Constant96/1 -> Goto257/1
  Constant97/1 -> Goto248/1
  Constant95/1 -> Goto253/1
  试一下增大1/1 -> Goto254/1
  Constant92/1 -> Goto263/1
  Constant93/1 -> Goto260/1
  Constant91/1 -> Goto258/1
  Constant90/1 -> Goto261/1
  Constant89/1 -> Goto249/1
  Constant88/1 -> Goto250/1
  Constant87/1 -> Goto246/1
  调大这个可以降低正输入，增大负输入2/1 -> Goto255/1
  调大这个可以抑制突变，但是会增大输入绝对值2/1 -> Goto241/1
  Constant84/1 -> Goto240/1
  Constant85/1 -> Goto243/1
  Constant86/1 -> Goto242/1
  Constant83/1 -> Goto244/1
  Constant82/1 -> Goto245/1
  Constant80/1 -> Goto256/1
  Constant81/1 -> Goto247/1
  Constant79/1 -> Goto251/1
  Constant78/1 -> Goto252/1
  Constant77/1 -> Goto262/1
  Constant98/1 -> Goto259/1
  From858/1 -> Integrator51/1
  pi/6→pi/2/1 -> Goto288/1
  From864/1 -> Product56/1
  Product59/1 -> Add26/1
  From865/1 -> Product56/2
  Cos25/1 -> Product66/2
  Cos24/1 -> Product63/2
  From876/1 -> Sin30/1
  From881/1 -> Product65/2
  Sin30/1 -> Product60/3
  From898/1 -> Product68/1
  Cos23/1 -> Product62/2
  From869/1 -> Integrator62/1
  Sin25/1 -> Product68/3
  From902/1 -> Integrator65/1
  Integrator61/1 -> Goto275/1, To Workspace27/1
  Sin31/1 -> Product65/3
  Product55/1 -> Add32/2
  From901/1 -> Cos20/1
  From859/1 -> Integrator53/1, Display35/1
  Integrator65/1 -> Goto267/1
  Cos21/1 -> Product58/2
  Integrator66/1 -> To Workspace31/1, Goto281/1
  From866/1 -> Sin28/1
  From885/1 -> Product64/2
  Constant99/1 -> Goto304/1
  -3→1/1 -> To Workspace33/1, Goto285/1
  From878/1 -> Cos24/1
  Integrator62/1 -> Scope63/1, Goto277/1, Product62/1
  From880/1 -> Integrator68/1
  From871/1 -> Product61/2
  From886/1 -> Sin32/1
  Product60/1 -> Add28/2
  From875/1 -> Product60/2
  From861/1 -> Product57/2
  From887/1 -> Cos25/1
  Product63/1 -> Add28/1
  From888/1 -> Cos26/1
  Integrator67/1 -> Product66/1, Goto283/1
  Add28/1 -> Integrator66/1
  From892/1 -> pi/6→pi/2/1
  From873/1 -> Product63/1
  From882/1 -> Sin31/1
  Sin29/1 -> Product61/3
  Integrator68/1 -> Goto284/1, Product65/1
  Product65/1 -> Add29/2
  From883/1 -> Product67/1
  Product62/1 -> Add27/1
  Product61/1 -> Add27/2
  Integrator63/1 -> To Workspace30/1, Goto276/1
  From874/1 -> Product60/1
  From884/1 -> Product64/1
  Product67/1 -> Add30/1
  Product66/1 -> Add29/1
  From897/1 -> Sin26/1
  Add32/1 -> Integrator60/1
  From872/1 -> Sin29/1
  Sin28/1 -> Product56/3
  From862/1 -> Sin27/1
  Integrator69/1 -> Goto286/1
  From860/1 -> Display34/1, Integrator57/1
  Product68/1 -> Add31/2
  Integrator56/1 -> To Workspace28/1, Goto264/1
  Clock8/1 -> MATLAB Function16/2(t)
  Integrator53/1 -> Product58/1, Goto273/1
  Product56/1 -> Add26/2
  From863/1 -> Product59/1
  Product70/1 -> Add32/1
  From889/1 -> Integrator69/1
  From899/1 -> Cos19/1
  Cos19/1 -> Product69/2
  From895/1 -> Product55/1
  Add31/1 -> Integrator56/1
  From891/1 -> Integrator70/1
  Add25/1 -> Integrator55/1
  Cos22/1 -> Product59/2
  From896/1 -> Product55/2
  MATLAB Function16/1(y) -> Goto270/1, Scope62/1
  From868/1 -> Cos22/1
  Integrator70/1 -> Goto287/1
  Product58/1 -> Add25/1
  Cos20/1 -> Product70/2
  Sin26/1 -> Product55/3
  Product57/1 -> Add25/2
  -14→-1/1 -> To Workspace32/1, Goto282/1
  Integrator64/1 -> Product61/1, Goto278/1
  Integrator57/1 -> Product57/1, Goto274/1
  Sin32/1 -> Product64/3
  From879/1 -> Integrator67/1
  Add26/1 -> Integrator61/1
  Product69/1 -> Add31/1
  Integrator60/1 -> To Workspace29/1, Goto266/1
  From870/1 -> Integrator64/1
  From900/1 -> MATLAB Function16/1(ks)
  From877/1 -> Cos23/1
  Add29/1 -> -14→-1/1
  From893/1 -> Sin25/1
  Add27/1 -> Integrator63/1
  Integrator55/1 -> To Workspace26/1, Goto272/1, Display33/1
  Integrator51/1 -> Goto265/1, Product69/1
  Add30/1 -> -3→1/1
  Sin27/1 -> Product57/3
  From867/1 -> Cos21/1
  From890/1 -> Product68/2
  Product64/1 -> Add30/2
  Cos26/1 -> Product67/2
  From894/1 -> Product70/1
  Constant118/1 -> Goto322/1
  Constant119/1 -> Goto313/1
  Constant117/1 -> Goto318/1
  试一下增大2/1 -> Goto319/1
  Constant115/1 -> Goto328/1
  Constant116/1 -> Goto325/1
  Constant114/1 -> Goto323/1
  Constant113/1 -> Goto326/1
  Constant112/1 -> Goto314/1
  Constant111/1 -> Goto315/1
  Constant110/1 -> Goto311/1
  调大这个可以降低正输入，增大负输入3/1 -> Goto320/1
  调大这个可以抑制突变，但是会增大输入绝对值3/1 -> Goto306/1
  Constant107/1 -> Goto305/1
  Constant108/1 -> Goto308/1
  Constant109/1 -> Goto307/1
  Constant106/1 -> Goto309/1
  Constant105/1 -> Goto310/1
  Constant103/1 -> Goto321/1
  Constant104/1 -> Goto312/1
  Constant102/1 -> Goto316/1
  Constant101/1 -> Goto317/1
  Constant100/1 -> Goto327/1
  Constant120/1 -> Goto324/1
  [theta1] -> Sin36/1
  Sin34/1 -> Product71/3
  [omgL] -> Product71/1
  Sin36/1 -> Product72/3
  Add44/1 -> -3→2/1
  Cos27/1 -> Product85/2
  [omg2] -> Integrator86/1
  Product75/1 -> Add34/1
  Integrator81/1 -> [thetaL]
  [dvL] -> Integrator71/1
  Cos37/1 -> Product78/2
  Integrator73/1 -> To Workspace34/1, [x1], Display36/1
  Cos36/1 -> Product75/2
  [dv3] -> Integrator83/1
  [h] -> Product76/2
  Product81/1 -> Add43/2
  [theta1] -> Cos35/1
  Product84/1 -> Add45/2
  [h] -> Product71/2
  Cos40/1 -> Product83/2
  Product80/1 -> Add44/2
  [vL] -> Product86/1
  Sin35/1 -> Product73/3
  [domg3] -> Integrator84/1
  Integrator71/1 -> [vL], Product85/1
  [h] -> Product84/2
  [ks] -> MATLAB Function17/1(ks)
  Integrator84/1 -> [omg3], Product81/1
  [theta3] -> Cos39/1
  Add35/1 -> -8.66025/1
  [omg1] -> Product72/1
  [theta2] -> Cos37/1
  [domg2] -> Integrator80/1
  [h] -> Product80/2
  [omg3] -> Product80/1
  [theta2] -> Sin38/1
  [v2] -> Product79/1
  [dv1] -> Integrator72/1, Display38/1
  Integrator76/1 -> To Workspace37/1, [yL]
  [theta3] -> Cos40/1
  [theta3] -> Sin40/1
  Product78/1 -> Add35/1
  Add34/1 -> Integrator77/1
  Sin40/1 -> Product80/3
  Product85/1 -> Add45/1
  Cos34/1 -> Product86/2
  Integrator75/1 -> Product73/1, [omg1]
  Add43/1 -> -25/1
  -8.66025/1 -> To Workspace38/1, [x2]
  Integrator80/1 -> Product77/1, Mux29/2, [omg2]  "omg2"
  Add46/1 -> Integrator76/1
  Product73/1 -> Add33/2
  Product74/1 -> Add33/1
  [theta1] -> Cos36/1
  MATLAB Function17/1(y) -> [omgL], Scope66/1
  Add45/1 -> Integrator74/1
  Add33/1 -> Integrator73/1
  [thetaL] -> Cos27/1
  [h] -> Product77/2
  Product86/1 -> Add46/1
  [v1] -> Product75/1
  Clock9/1 -> MATLAB Function17/2(t)
  Integrator77/1 -> [y1], To Workspace35/1
  Integrator74/1 -> To Workspace36/1, [xL]
  Product77/1 -> Add35/2
  Integrator72/1 -> Product74/1, [v1]
  Cos39/1 -> Product82/2
  [thetaL] -> Sin34/1
  [theta2] -> Sin37/1
  [omg1] -> Integrator85/1
  [theta1] -> Sin35/1
  [h] -> Product73/2
  [theta3] -> Sin39/1
  [v3] -> Product83/1
  Sin37/1 -> Product77/3
  [omg3] -> pi/9/1
  Add42/1 -> Integrator82/1
  [thetaL] -> Sin33/1
  Cos38/1 -> Product79/2
  Integrator83/1 -> Product82/1, [v3]
  Product79/1 -> Add42/1
  Product72/1 -> Add34/2
  [theta2] -> Cos38/1
  Integrator86/1 -> [theta2]
  Product76/1 -> Add42/2
  Cos35/1 -> Product74/2
  Product82/1 -> Add43/1
  pi/9/1 -> [theta3]
  -3→2/1 -> To Workspace41/1, [y3]
  -25/1 -> To Workspace40/1, [x3]
  Integrator78/1 -> Mux29/1, [v2], Product78/1  "v2"
  [omg2] -> Product76/1
  Integrator85/1 -> [theta1]
  Integrator82/1 -> To Workspace39/1, [y2]
  Sin39/1 -> Product81/3
  [domg1] -> Display37/1, Integrator75/1
  [thetaL] -> Cos34/1
  Product71/1 -> Add46/2
  Sin38/1 -> Product76/3
  Product83/1 -> Add44/1
  [omgL] -> Integrator81/1
  [h] -> Product81/2
  [dv2] -> Integrator78/1
  [h] -> Product72/2
  [omgL] -> Product84/1
  Sin33/1 -> Product84/3
  Constant24/1 -> Goto348/1
  Constant61/1 -> Goto331/1
  Constant58/1 -> Goto337/1
  试一下增大3/1 -> Goto340/1
  Constant73/1 -> Goto339/1
  Constant66/1 -> Goto332/1
  调大这个可以降低正输入，增大负输入1/1 -> Goto341/1
  Constant70/1 -> Goto344/1
  Constant57/1 -> Goto338/1
  Constant65/1 -> Goto220/1
  Constant60/1 -> Goto333/1
  Constant59/1 -> Goto342/1
  Constant76/1 -> Goto345/1
  Constant64/1 -> Goto329/1
  Constant67/1 -> Goto336/1
  Constant62/1 -> Goto330/1
  调大这个可以抑制突变，但是会增大输入绝对值1/1 -> Goto219/1
  Constant68/1 -> Goto335/1
  Constant74/1 -> Goto343/1
  Constant72/1 -> Goto346/1
  Constant71/1 -> Goto349/1
  Constant63/1 -> Goto218/1
  Constant69/1 -> Goto347/1
  Constant75/1 -> Goto334/1
  MATLAB Function18/1(y) -> Scope99/1, [rphi23]
  Mux29/1 -> Scope67/1
  Constant121/1 -> Scope69/1, [lowz3p]
  Constant143/1 -> Goto358/1
  Constant136/1 -> Goto371/1
  Constant129/1 -> Goto350/1
  Constant139/1 -> Goto373/1
  Constant140/1 -> Goto370/1
  Constant142/1 -> Goto367/1
  Constant135/1 -> Goto359/1
  调大这个可以抑制突变，但是会增大输入绝对值4/1 -> Goto351/1
  Constant128/1 -> Goto354/1
  Constant134/1 -> Goto360/1
  Constant130/1 -> Goto353/1
  Constant148/1 -> Goto369/1
  Constant125/1 -> Goto366/1
  Constant126/1 -> Goto357/1
  Constant131/1 -> Goto352/1
  Constant123/1 -> Goto362/1
  Constant137/1 -> Goto368/1
  调大这个可以降低正输入，增大负输入4/1 -> Goto365/1
  Constant132/1 -> Goto356/1
  Constant141/1 -> Goto363/1
  试一下增大4/1 -> Goto364/1
  Constant124/1 -> Goto361/1
  Constant127/1 -> Goto355/1
  Constant122/1 -> Goto372/1
  Constant149/1 -> Goto396/1
  Constant154/1 -> Goto379/1
  Constant151/1 -> Goto385/1
  越大phip超调越大/1 -> Goto388/1
  越大phid超调越大/1 -> Goto387/1
  Constant159/1 -> Goto380/1
  调大这个可以降低正输入，增大负输入5/1 -> Goto389/1
  Constant163/1 -> Goto392/1
  Constant150/1 -> Goto386/1
  Constant158/1 -> Goto376/1
  Constant153/1 -> Goto381/1
  Constant152/1 -> Goto390/1
  Constant169/1 -> Goto393/1
  Constant157/1 -> Goto377/1
  Constant160/1 -> Goto384/1
  Constant155/1 -> Goto378/1
  调大这个可以抑制突变，但是会增大输入绝对值5/1 -> Goto375/1
  Constant161/1 -> Goto383/1
  Constant167/1 -> Goto391/1
  Constant165/1 -> Goto394/1
  Constant164/1 -> Goto397/1
  Constant156/1 -> Goto374/1
  Constant162/1 -> Goto395/1
  Constant168/1 -> Goto382/1
  MATLAB Function5/1(tauiL) -> Saturation6/1
  Saturation6/1 -> Mux21/1, Display20/1, Mux32/3, [tau3L]  "tau3L"
  MATLAB Function6/1(tauiR) -> Saturation7/1
  Saturation7/1 -> Display21/1, Mux33/3, Mux21/2, [tau3R]  "tau3R"
  Constant187/1 -> Goto406/1
  Constant182/1 -> Goto419/1
  Constant176/1 -> Goto398/1
  Constant184/1 -> Goto421/1
  Constant185/1 -> Goto418/1
  Constant186/1 -> Goto415/1
  Constant181/1 -> Goto407/1
  调大这个可以抑制突变，但是会增大输入绝对值6/1 -> Goto399/1
  Constant175/1 -> Goto402/1
  Constant180/1 -> Goto408/1
  Constant177/1 -> Goto401/1
  Constant188/1 -> Goto417/1
  Constant172/1 -> Goto414/1
  Constant173/1 -> Goto405/1
  Constant178/1 -> Goto400/1
  Constant170/1 -> Goto410/1
  Constant183/1 -> Goto416/1
  调大这个可以降低正输入，增大负输入6/1 -> Goto413/1
  Constant179/1 -> Goto404/1
  越大phid超调越大1/1 -> Goto411/1
  越大phip超调越大1/1 -> Goto412/1
  Constant171/1 -> Goto409/1
  Constant174/1 -> Goto403/1
  Constant166/1 -> Goto420/1
  Constant189/1 -> Goto444/1
  Constant194/1 -> Goto427/1
  Constant191/1 -> Goto433/1
  越大phip超调越大2/1 -> Goto436/1
  越大phid超调越大2/1 -> Goto435/1
  Constant199/1 -> Goto428/1
  调大这个可以降低正输入，增大负输入7/1 -> Goto437/1
  Constant203/1 -> Goto440/1
  Constant190/1 -> Goto434/1
  Constant198/1 -> Goto424/1
  Constant193/1 -> Goto429/1
  Constant192/1 -> Goto438/1
  Constant208/1 -> Goto441/1
  Constant197/1 -> Goto425/1
  Constant200/1 -> Goto432/1
  Constant195/1 -> Goto426/1
  调大这个可以抑制突变，但是会增大输入绝对值7/1 -> Goto423/1
  Constant201/1 -> Goto431/1
  Constant206/1 -> Goto439/1
  Constant205/1 -> Goto442/1
  Constant204/1 -> Goto445/1
  Constant196/1 -> Goto422/1
  Constant202/1 -> Goto443/1
  Constant207/1 -> Goto430/1
  Constant227/1 -> Goto454/1
  Constant222/1 -> Goto467/1
  Constant216/1 -> Goto446/1
  Constant224/1 -> Goto469/1
  Constant225/1 -> Goto466/1
  Constant226/1 -> Goto463/1
  Constant221/1 -> Goto455/1
  调大这个可以抑制突变，但是会增大输入绝对值8/1 -> Goto447/1
  Constant215/1 -> Goto450/1
  Constant220/1 -> Goto456/1
  Constant217/1 -> Goto449/1
  Constant228/1 -> Goto465/1
  Constant212/1 -> Goto462/1
  Constant213/1 -> Goto453/1
  Constant218/1 -> Goto448/1
  Constant210/1 -> Goto458/1
  Constant223/1 -> Goto464/1
  调大这个可以降低正输入，增大负输入8/1 -> Goto461/1
  Constant219/1 -> Goto452/1
  越大phid超调越大3/1 -> Goto459/1
  越大phip超调越大3/1 -> Goto460/1
  Constant211/1 -> Goto457/1
  Constant214/1 -> Goto451/1
  Constant209/1 -> Goto468/1
  Mux30/1 -> Scope72/1
  Sin41/1 -> Product102/3
  From995/1 -> Product102/1
  From961/1 -> Product88/2
  From965/1 -> Integrator94/1
  From977/1 -> Product99/2
  From999/1 -> Integrator97/1
  Product101/1 -> Add52/1
  Sin46/1 -> Product92/3
  Product87/1 -> Add54/2
  From998/1 -> Cos42/1
  From952/1 -> Integrator91/1, Display40/1
  Sin47/1 -> Product99/3
  Integrator98/1 -> Goto480/1, To Workspace47/1
  Integrator101/1 -> Goto485/1
  From970/1 -> Product92/1
  Integrator94/1 -> Product94/1, Goto478/1, Mux30/1  "v2"
  -14→-3/1 -> Goto481/1, To Workspace48/1
  -3→3/1 -> Goto484/1, To Workspace50/1
  " "/1 -> Goto487/1
  Product100/1 -> Add51/1
  Cos43/1 -> Product90/2
  Product92/1 -> Add50/2
  Integrator102/1 -> Goto486/1
  From974/1 -> Cos46/1
  Product88/1 -> Add48/2
  Product97/1 -> Add50/1
  Integrator99/1 -> Goto482/1, Product100/1
  Cos46/1 -> Product97/2
  From989/1 -> Sin41/1
  Add50/1 -> Integrator98/1
  From988/1 -> " "/1
  Sin45/1 -> Product93/3
  From979/1 -> Product101/1
  From978/1 -> Sin47/1
  From953/1 -> Product89/2
  From954/1 -> Sin43/1
  From985/1 -> Integrator101/1
  From968/1 -> Sin45/1
  From994/1 -> Sin42/1
  Cos47/1 -> Product100/2
  Integrator88/1 -> Goto474/1, Product90/1
  Product93/1 -> Add49/2
  Integrator90/1 -> Goto489/1, To Workspace44/1
  Integrator93/1 -> To Workspace43/1, Goto476/1
  From955/1 -> Product91/1
  Product104/1 -> Add54/1
  From967/1 -> Product93/2
  From996/1 -> Cos41/1
  Add47/1 -> Integrator89/1
  Add53/1 -> Integrator90/1
  From964/1 -> Cos44/1
  Product90/1 -> Add47/1
  Product89/1 -> Add47/2
  Add54/1 -> Integrator92/1
  Integrator96/1 -> Goto479/1, Mux30/2, Product93/1  "omg2"
  Integrator95/1 -> Goto477/1, To Workspace46/1
  Add51/1 -> -14→-3/1
  Integrator91/1 -> Goto475/1, Product89/1
  Cos42/1 -> Product104/2
  Product103/1 -> Add53/1
  Sin48/1 -> Product98/3
  Add48/1 -> Integrator93/1
  Product94/1 -> Add49/1
  From982/1 -> Sin48/1
  From984/1 -> Cos48/1
  Integrator92/1 -> Goto470/1, To Workspace45/1
  From951/1 -> Display42/1, Integrator88/1
  From969/1 -> Product97/1
  From972/1 -> Sin46/1
  From980/1 -> Product98/1
  From981/1 -> Product98/2
  From966/1 -> Integrator96/1
  From973/1 -> Cos45/1
  From956/1 -> Product88/1
  Add49/1 -> Integrator95/1
  From983/1 -> Cos47/1
  Integrator100/1 -> Product99/1, Goto483/1
  From986/1 -> Product102/2
  Integrator87/1 -> Product103/1, Goto490/1
  From976/1 -> Integrator100/1
  Sin43/1 -> Product89/3
  From990/1 -> Product104/1
  Product98/1 -> Add52/2
  Cos48/1 -> Product101/2
  From992/1 -> Product87/2
  Product102/1 -> Add53/2
  From963/1 -> Cos43/1
  Product99/1 -> Add51/2
  From971/1 -> Product92/2
  From975/1 -> Integrator99/1
  Cos44/1 -> Product91/2
  Integrator89/1 -> Display39/1, Goto473/1, To Workspace42/1
  Cos45/1 -> Product94/2
  From950/1 -> Integrator87/1
  Integrator97/1 -> Goto471/1
  Product91/1 -> Add48/1
  From987/1 -> Integrator102/1
  Cos41/1 -> Product103/2
  Add52/1 -> -3→3/1
  Sin44/1 -> Product88/3
  From991/1 -> Product87/1
  Sin42/1 -> Product87/3
  From962/1 -> Sin44/1
  alpha1/1(y) -> Scope71/1, Goto472/1
  Clock10/1 -> alpha1/1(t)
  Constant229/1 -> Goto512/1
  Constant234/1 -> Goto495/1
  Constant231/1 -> Goto501/1
  越大phip超调越大4/1 -> Goto504/1
  越大phid超调越大4/1 -> Goto503/1
  Constant239/1 -> Goto496/1
  调大这个可以降低正输入，增大负输入9/1 -> Goto505/1
  Constant243/1 -> Goto508/1
  Constant230/1 -> Goto502/1
  Constant238/1 -> Goto492/1
  Constant233/1 -> Goto497/1
  Constant232/1 -> Goto506/1
  Constant248/1 -> Goto509/1
  Constant237/1 -> Goto493/1
  Constant240/1 -> Goto500/1
  Constant235/1 -> Goto494/1
  调大这个可以抑制突变，但是会增大输入绝对值9/1 -> Goto491/1
  Constant241/1 -> Goto499/1
  Constant246/1 -> Goto507/1
  Constant245/1 -> Goto510/1
  Constant244/1 -> Goto513/1
  Constant236/1 -> Goto488/1
  Constant242/1 -> Goto511/1
  Constant247/1 -> Goto498/1
  Constant250/1 -> Goto12/1
  Constant35/1 -> Goto40/1
  Constant11/1 -> Goto1/1
  Constant43/1 -> Goto42/1
  Constant94/1 -> Goto39/1
  Constant249/1 -> Goto36/1
  Constant34/1 -> Goto13/1
  调大这个可以抑制突变，但是会增大输入绝对值10/1 -> Goto5/1
  Constant10/1 -> Goto8/1
  Constant15/1 -> Goto14/1
  Constant12/1 -> Goto7/1
  Constant251/1 -> Goto38/1
  Constant6/1 -> Goto35/1
  Constant8/1 -> Goto11/1
  Constant13/1 -> Goto6/1
  Constant2/1 -> Goto24/1
  Constant42/1 -> Goto37/1
  调大这个可以降低正输入，增大负输入10/1 -> Goto34/1
  Constant14/1 -> Goto10/1
  越大phid超调越大5/1 -> Goto29/1
  越大phip超调越大5/1 -> Goto33/1
  Constant5/1 -> Goto15/1
  Constant9/1 -> Goto9/1
  Constant1/1 -> Goto41/1
  Saturation8/1 -> Mux20/1, Mux32/2, [tau2L]  "tau2L"
  Saturation9/1 -> Mux20/2, Display25/1, Mux33/2, [tau2R]  "tau2R"
  Mux19/1 -> Scope44/1
  Saturation10/1 -> Mux19/1, Display16/1, Mux32/1, [tau1L]  "tau1L"
  Saturation11/1 -> Mux33/1, [tau1R], Mux19/2, Display17/1  "tau1R"
  Constant252/1 -> [k1roup]
  Constant257/1 -> [k3p]
  Constant254/1 -> [D1dm]
  越大phip超调越大6/1 -> [D3pm]
  越大phid超调越大6/1 -> [D3dm]
  Constant262/1 -> [k2ed]
  调大这个可以降低正输入，增大负输入11/1 -> [k2ep]
  Constant266/1 -> [k2roud]
  Constant253/1 -> [D1pm]
  Constant261/1 -> [k1d]
  Constant256/1 -> [k1ed]
  Constant255/1 -> [k1ep]
  Constant271/1 -> [k1roud]
  Constant260/1 -> [k1p]
  Constant263/1 -> [D2pm]
  Constant258/1 -> [k3d]
  调大这个可以抑制突变，但是会增大输入绝对值11/1 -> [k2p]
  Constant264/1 -> [D2dm]
  Constant269/1 -> [k3ep]
  Constant268/1 -> [k3roud]
  Constant267/1 -> [k3roup]
  Constant259/1 -> [k2d]
  Constant265/1 -> [k2roup]
  Constant270/1 -> [k3ed]
  Integrator/1 -> Mux26/1, Scope5/1, MATLAB Function/3(Didm_hat), [D1dm_hat]  "D1dm_hat"
  MATLAB Function/1(y) -> Integrator/1  "dot D1dm_hat"
  [delta11] -> MATLAB Function/4(delta_id)
  Constant272/1 -> MATLAB Function/2(sigma_id)
  Constant273/1 -> MATLAB Function/1(gamma_id)
  Constant275/1 -> MATLAB Function9/1(gamma_id)
  Constant274/1 -> MATLAB Function9/2(sigma_id)
  [delta21] -> MATLAB Function9/4(delta_id)
  MATLAB Function9/1(y) -> Integrator1/1  "dot D2dm_hat"
  Integrator1/1 -> Mux26/2, MATLAB Function9/3(Didm_hat), [D2dm_hat], Scope6/1  "D2dm_hat"
  Integrator2/1 -> Mux26/3, Scope7/1, MATLAB Function33/3(Didm_hat), [D3dm_hat]  "D3dm_hat"
  MATLAB Function33/1(y) -> Integrator2/1  "dot D3dm_hat"
  [delta31] -> MATLAB Function33/4(delta_id)
  Constant276/1 -> MATLAB Function33/2(sigma_id)
  Constant277/1 -> MATLAB Function33/1(gamma_id)
  Constant279/1 -> MATLAB Function34/1(gamma_id)
  Constant278/1 -> MATLAB Function34/2(sigma_id)
  [delta12] -> MATLAB Function34/4(delta_id)
  MATLAB Function34/1(y) -> Integrator3/1  "dot D1pm_hat"
  Integrator3/1 -> Mux31/1, MATLAB Function34/3(Didm_hat), [D1pm_hat], Scope8/1  "D1pm_hat"
  Integrator4/1 -> Mux31/2, Scope15/1, MATLAB Function35/3(Didm_hat), [D2pm_hat]  "D2pm_hat"
  MATLAB Function35/1(y) -> Integrator4/1  "dot D2pm_hat"
  [delta22] -> MATLAB Function35/4(delta_id)
  Constant280/1 -> MATLAB Function35/2(sigma_id)
  Constant281/1 -> MATLAB Function35/1(gamma_id)
  Constant283/1 -> MATLAB Function36/1(gamma_id)
  Constant282/1 -> MATLAB Function36/2(sigma_id)
  [delta32] -> MATLAB Function36/4(delta_id)
  MATLAB Function36/1(y) -> Integrator5/1  "dot D3pm_hat"
  Integrator5/1 -> Mux31/3, MATLAB Function36/3(Didm_hat), [D3pm_hat], Scope16/1  "D3pm_hat"
  [delta11] -> u1d/5(deltaid)
  [delta12] -> u1p/5(deltaip)
  Constant302/1 -> Goto290/1
  Constant297/1 -> Goto124/1
  Constant291/1 -> Goto127/1
  Constant299/1 -> Goto126/1
  Constant300/1 -> Goto123/1
  Constant301/1 -> Goto299/1
  Constant296/1 -> Goto291/1
  调大这个可以抑制突变，但是会增大输入绝对值12/1 -> Goto128/1
  Constant290/1 -> Goto131/1
  Constant295/1 -> Goto292/1
  Constant292/1 -> Goto130/1
  Constant303/1 -> Goto122/1
  Constant287/1 -> Goto298/1
  Constant288/1 -> Goto289/1
  Constant293/1 -> Goto129/1
  Constant285/1 -> Goto294/1
  Constant298/1 -> Goto300/1
  调大这个可以降低正输入，增大负输入12/1 -> Goto297/1
  Constant294/1 -> Goto198/1
  越大phid超调越大7/1 -> Goto295/1
  越大phip超调越大7/1 -> Goto296/1
  Constant286/1 -> Goto293/1
  Constant289/1 -> Goto132/1
  Constant284/1 -> Goto125/1
  Constant304/1 -> [ked]
  Constant305/1 -> [kep]
  Mux26/1 -> Didm_hat/1
  Mux31/1 -> Dipm_hat/1
  Constant306/1 -> Goto530/1
  Constant324/1 -> Goto536/1
  Constant321/1 -> Goto519/1
  越大phip超调越大8/1 -> Goto522/1
  越大phid超调越大8/1 -> Goto521/1
  Constant311/1 -> Goto514/1
  调大这个可以降低正输入，增大负输入13/1 -> Goto523/1
  Constant319/1 -> Goto526/1
  Constant313/1 -> Goto520/1
  Constant310/1 -> Goto533/1
  Constant323/1 -> Goto515/1
  Constant322/1 -> Goto524/1
  Constant316/1 -> Goto527/1
  Constant309/1 -> Goto534/1
  Constant312/1 -> Goto518/1
  Constant307/1 -> Goto535/1
  调大这个可以抑制突变，但是会增大输入绝对值13/1 -> Goto532/1
  Constant317/1 -> Goto517/1
  Constant314/1 -> Goto525/1
  Constant325/1 -> Goto528/1
  Constant320/1 -> Goto531/1
  Constant308/1 -> Goto303/1
  Constant318/1 -> Goto529/1
  Constant315/1 -> Goto516/1
  原常数/1 -> [ks]
  原常数1/1 -> Goto538/1
  Clock4/1 -> MATLAB Function37/2(t)
  MATLAB Function37/1(y) -> Scope20/1, Goto537/1
  From2/1 -> MATLAB Function37/1(ks)
  Mux32/1 -> To Workspace10/1, tauiL/1
  Mux33/1 -> To Workspace11/1, tauiR/1
  [M] -> a5/6(m)
  [J] -> a6/4(j)
  [arfL2] -> a4/1(a)
  a5/1(y) -> Display2/1, [bb2]
  [M] -> a6/6(m)
  [l] -> a6/3(l)
  [J] -> a5/4(j)
  [J] -> a7/4(j)
  [h] -> a7/2(h)
  a7/1(y) -> Display4/1, [cc2]
  [J] -> a4/4(j)
  [h] -> a6/2(h)
  [r] -> a4/5(r)
  [h] -> a4/2(h)
  [l] -> a5/3(l)
  [l] -> a4/3(l)
  [r] -> a5/5(r)
  a6/1(y) -> Display3/1, [dd2]
  [M] -> a4/6(m)
  [M] -> a7/6(m)
  [arfL2] -> a7/1(a)
  [h] -> a5/2(h)
  [arfL2] -> a6/1(a)
  [arfL2] -> a5/1(a)
  [r] -> a6/5(r)
  [l] -> a7/3(l)
  [r] -> a7/5(r)
  a4/1(y) -> Display1/1, [aa2]
  [aa2] -> MATLAB Function32/1(aa)
  [cc2] -> MATLAB Function32/3(cc)
  [dd2] -> MATLAB Function32/4(dd)
  [bb2] -> MATLAB Function32/2(bb)
  [l] -> a11/3(l)
  a8/1(y) -> Display5/1, [aa3]
  [r] -> a11/5(r)
  [arf23] -> a9/1(a)
  [r] -> a10/5(r)
  [h] -> a10/2(h)
  [r] -> a8/5(r)
  [r] -> a9/5(r)
  [arf23] -> a10/1(a)
  [M] -> a8/6(m)
  [l] -> a8/3(l)
  [h] -> a9/2(h)
  [arf23] -> a11/1(a)
  [J] -> a8/4(j)
  a10/1(y) -> Display7/1, [dd3]
  [M] -> a11/6(m)
  [M] -> a10/6(m)
  [l] -> a10/3(l)
  [h] -> a11/2(h)
  [J] -> a11/4(j)
  [J] -> a10/4(j)
  [J] -> a9/4(j)
  [l] -> a9/3(l)
  [h] -> a8/2(h)
  a11/1(y) -> Display8/1, [cc3]
  [M] -> a9/6(m)
  a9/1(y) -> Display6/1, [bb3]
  [arf23] -> a8/1(a)
  [aa3] -> MATLAB Function6/1(aa)
  [cc3] -> MATLAB Function6/3(cc)
  [dd3] -> MATLAB Function6/4(dd)
  [bb3] -> MATLAB Function6/2(bb)
  From166/1 -> Cos6/1
  From278/1 -> Product32/1
  Sin6/1 -> Product24/3
  Sin7/1 -> Product29/3
  -1/1 -> To Workspace7/1, Goto558/1
  Cos4/1 -> Product23/2
  Sin2/1 -> Product1/3
  From271/1 -> Integrator20/1
  Product23/1 -> Add6/1
  Product32/1 -> Add11/2
  Cos5/1 -> Product26/2
  Product29/1 -> Add9/2
  Cos1/1 -> Product33/2
  Add10/1 -> -3→4/1
  Sin4/1 -> Product2/3
  From275/1 -> Product1/1
  Cos2/1 -> Product34/2
  From252/1 -> Cos8/1
  -8.1/1 -> To Workspace5/1, Goto554/1
  From247/1 -> Sin8/1
  Integrator11/1 -> To Workspace4/1, Goto547/1
  From165/1 -> Cos5/1
  From208/1 -> Integrator18/1
  Integrator6/1 -> Goto567/1, Product33/1
  Cos8/1 -> Product31/2
  Integrator18/1 -> Goto560/1, Product29/1
  Integrator15/1 -> Goto548/1
  Product28/1 -> Add10/2
  From251/1 -> Cos7/1
  Integrator10/1 -> Product3/1, Goto552/1
  Add6/1 -> Integrator12/1
  From163/1 -> Product24/2
  From144/1 -> Sin4/1
  Cos7/1 -> Product30/2
  Sin3/1 -> Product3/3
  Integrator13/1 -> Mux34/1, Goto555/1, Product26/1  "v2"
  原常数2/1 -> Goto565/1
  From137/1 -> Display10/1, Integrator10/1
  From145/1 -> Cos3/1
  From245/1 -> Product28/1
  From273/1 -> Sin1/1
  Clock5/1 -> MATLAB Function38/1(t)
  From241/1 -> Product29/2
  From242/1 -> Sin7/1
  From142/1 -> Product2/1
  Sin8/1 -> Product28/3
  Add5/1 -> Integrator8/1
  Add7/1 -> -8.1/1
  Integrator14/1 -> Product25/1, Mux34/2, Goto556/1  "omg2"
  From282/1 -> Integrator15/1
  Product33/1 -> Add11/1
  -3→4/1 -> To Workspace8/1, Goto561/1
  From162/1 -> Product24/1
  Integrator16/1 -> To Workspace6/1, Goto557/1
  Product1/1 -> Add13/2
  Integrator7/1 -> Product4/1, Goto551/1
  Product27/1 -> Add8/1
  Sin5/1 -> Product25/3
  From243/1 -> Product31/1
  Product25/1 -> Add7/2
  From159/1 -> Product25/2
  Product34/1 -> Add13/1
  Integrator9/1 -> To Workspace3/1, Goto566/1
  From269/1 -> Integrator19/1
  From140/1 -> Sin3/1
  From139/1 -> Product3/2
  From160/1 -> Sin5/1
  Add13/1 -> Integrator11/1
  From146/1 -> Cos4/1
  MATLAB Function38/1(y) -> Goto549/1, Scope21/1
  Integrator20/1 -> Goto563/1
  From277/1 -> Sin2/1
  Product2/1 -> Add6/2
  From136/1 -> Integrator7/1, Display11/1
  Cos6/1 -> Product27/2
  Add8/1 -> Integrator16/1
  From279/1 -> Cos1/1
  Product4/1 -> Add5/1
  From272/1 -> pi/1/1
  Integrator12/1 -> Goto553/1, To Workspace2/1
  From281/1 -> Cos2/1
  Cos3/1 -> Product4/2
  From143/1 -> Product2/2
  From270/1 -> Product32/2
  From274/1 -> Product34/1
  Integrator8/1 -> To Workspace1/1, Goto550/1, Display9/1
  Product24/1 -> Add8/2
  Mux34/1 -> Scope22/1
  From161/1 -> Product27/1
  Add11/1 -> Integrator9/1
  From147/1 -> Integrator13/1
  Product30/1 -> Add9/1
  From164/1 -> Sin6/1
  From280/1 -> ?
  Product3/1 -> Add5/2
  Integrator19/1 -> Goto562/1
  From156/1 -> Integrator14/1
  Product26/1 -> Add7/1
  From167/1 -> Integrator17/1
  From134/1 -> Integrator6/1
  Product31/1 -> Add10/1
  pi/1/1 -> Goto564/1
  From276/1 -> Product1/2
  From141/1 -> Product23/1
  Sin1/1 -> Product32/3
  Add9/1 -> -1/1
  Integrator17/1 -> Product30/1, Goto559/1
  From246/1 -> Product28/2
